simulink model "AIRCRAFT_ENGINE"  (Simulink 7.3)
settings: Solver=ode45  StartTime=0.0  StopTime=10.0  RelTol=1e-3
undefined symbols (not defined in the file): RootGround, RootPart
libraries: mblibv1 x68
settings Model: Creator=alvarez3  LastModifiedBy=congyue1
settings SimMechanicsCC: VisOnUpdateDiagram=on  VisDuringSimulation=on

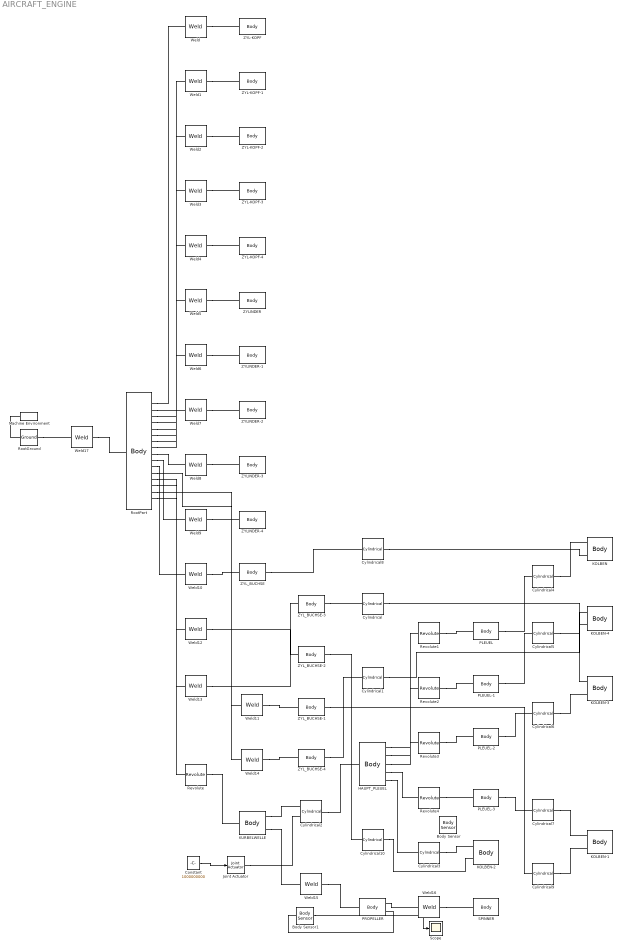
== system AIRCRAFT_ENGINE ==
  Body Sensor : mblibv1/Sensors &  Actuators/Body Sensor  DialogController=MECH.DynMechDlgSource  SystemSampleTime=-1  UpdateFromCAD=off  PhysicalDomain=Mechanical  PortType=blob  Muxed=on  Pose=off  Angle=on  AngleUnits=deg  ArcVelocity=off  ArcVelocityUnits=deg/s  ArcAcceleration=off  ArcAccelerationUnits=deg/s^2  CoordPosition=on  CoordPositionUnits=m  Velocity=off  VelocityUnits=m/s  Acceleration=off  AccelerationUnits=m/s^2  Quaternion=on  QuaternionDT=off  QuaternionDDT=off  QuaternionUnits=off  OutputVector=[1]  ActiveIO=off  Width=3  DialogClass=MechanicalSensorBlock  ReferenceFrame=Absolute (World)
  Body Sensor1 : mblibv1/Sensors &  Actuators/Body Sensor  DialogController=MECH.DynMechDlgSource  SystemSampleTime=-1  UpdateFromCAD=off  PhysicalDomain=Mechanical  PortType=blob  Muxed=on  Pose=on  Angle=on  AngleUnits=deg  ArcVelocity=off  ArcVelocityUnits=deg/s  ArcAcceleration=off  ArcAccelerationUnits=deg/s^2  CoordPosition=on  CoordPositionUnits=m  Velocity=off  VelocityUnits=m/s  Acceleration=off  AccelerationUnits=m/s^2  Quaternion=on  QuaternionDT=off  QuaternionDDT=off  QuaternionUnits=off  OutputVector=[1]  ActiveIO=on  Width=12  DialogClass=MechanicalSensorBlock  ReferenceFrame=Absolute (World)
  Constant : Constant  Value=1000000000  OutDataType=fixdt(1, 16)  OutScaling=2^0
  Cylindrical : mblibv1/Joints/Cylindrical  DialogController=MECH.DynMechDlgSource  PhysicalDomain=mechanical  SubClassName=Unknown  LeftPortType=blob  RightPortType=blob  LConnTagsString=__newl0  RConnTagsString=__newr0  PMImportedID=110:-:62  UpdateFromCAD=on  NumSAPorts=0  CutJoint=off  MarkAsCut=off  Primitives=prismatic  PrimitiveProps=P1$WORLD$[0,-0.309017,-0.951057]$prismatic#R1$WORLD$[0,0.309017,0.951057]$revolute  DialogClass=JointBlock  P1Axis=[0,-0.309017,-0.951057]  R1Axis=[0,0.309017,0.951057]
  Cylindrical1 : mblibv1/Joints/Cylindrical  DialogController=MECH.DynMechDlgSource  PhysicalDomain=mechanical  SubClassName=Unknown  LeftPortType=blob  RightPortType=blob  LConnTagsString=__newl0  RConnTagsString=__newr0  PMImportedID=81:-:89  UpdateFromCAD=on  NumSAPorts=0  CutJoint=off  MarkAsCut=off  Primitives=prismatic  PrimitiveProps=P1$WORLD$[0,0.809017,-0.587785]$prismatic#R1$WORLD$[0,-0.809017,0.587785]$revolute  DialogClass=JointBlock  P1Axis=[0,0.809017,-0.587785]  R1Axis=[0,-0.809017,0.587785]
  Cylindrical10 : mblibv1/Joints/Cylindrical  DialogController=MECH.DynMechDlgSource  PhysicalDomain=mechanical  SubClassName=Unknown  LeftPortType=blob  RightPortType=blob  LConnTagsString=__newl0  RConnTagsString=__newr0  PMImportedID=29:-:75  UpdateFromCAD=on  NumSAPorts=0  CutJoint=off  MarkAsCut=off  Primitives=prismatic  PrimitiveProps=P1$WORLD$[0,-0.309017,0.951057]$prismatic#R1$WORLD$[0,0.309017,-0.951057]$revolute  DialogClass=JointBlock  P1Axis=[0,-0.309017,0.951057]  R1Axis=[0,0.309017,-0.951057]
  Cylindrical2 : mblibv1/Joints/Cylindrical  DialogController=MECH.DynMechDlgSource  PhysicalDomain=mechanical  SubClassName=Unknown  LeftPortType=blob  RightPortType=blob  LConnTagsString=__newl0|SA1  RConnTagsString=__newr0  PMImportedID=74:-:76  UpdateFromCAD=on  NumSAPorts=1  CutJoint=off  MarkAsCut=off  Primitives=prismatic  PrimitiveProps=P1$World$[-1,0,0]$prismatic#R1$World$[1,0,0]$revolute  DialogClass=JointBlock  P1Axis=[-1,0,0]  R1Axis=[1,0,0]
  Cylindrical3 : mblibv1/Joints/Cylindrical  DialogController=MECH.DynMechDlgSource  PhysicalDomain=mechanical  SubClassName=Unknown  LeftPortType=blob  RightPortType=blob  LConnTagsString=__newl0  RConnTagsString=__newr0  PMImportedID=74:-:75  UpdateFromCAD=on  NumSAPorts=0  CutJoint=off  MarkAsCut=off  Primitives=prismatic  PrimitiveProps=P1$WORLD$[1,0,0]$prismatic#R1$WORLD$[-1,0,0]$revolute  DialogClass=JointBlock  P1Axis=[1,0,0]  R1Axis=[-1,0,0]
  Cylindrical4 : mblibv1/Joints/Cylindrical  DialogController=MECH.DynMechDlgSource  PhysicalDomain=mechanical  SubClassName=Unknown  LeftPortType=blob  RightPortType=blob  LConnTagsString=__newl0  RConnTagsString=__newr0  PMImportedID=106:-:79  UpdateFromCAD=on  NumSAPorts=0  CutJoint=off  MarkAsCut=off  Primitives=prismatic  PrimitiveProps=P1$WORLD$[1,0,0]$prismatic#R1$WORLD$[1,0,0]$revolute  DialogClass=JointBlock  P1Axis=[1,0,0]  R1Axis=[1,0,0]
  Cylindrical5 : mblibv1/Joints/Cylindrical  DialogController=MECH.DynMechDlgSource  PhysicalDomain=mechanical  SubClassName=Unknown  LeftPortType=blob  RightPortType=blob  LConnTagsString=__newl0  RConnTagsString=__newr0  PMImportedID=108:-:81  UpdateFromCAD=on  NumSAPorts=0  CutJoint=off  MarkAsCut=off  Primitives=prismatic  PrimitiveProps=P1$WORLD$[1,0,0]$prismatic#R1$WORLD$[-1,0,0]$revolute  DialogClass=JointBlock  P1Axis=[1,0,0]  R1Axis=[-1,0,0]
  Cylindrical6 : mblibv1/Joints/Cylindrical  DialogController=MECH.DynMechDlgSource  PhysicalDomain=mechanical  SubClassName=Unknown  LeftPortType=blob  RightPortType=blob  LConnTagsString=__newl0  RConnTagsString=__newr0  PMImportedID=110:-:113  UpdateFromCAD=on  NumSAPorts=0  CutJoint=off  MarkAsCut=off  Primitives=prismatic  PrimitiveProps=P1$WORLD$[1,0,0]$prismatic#R1$WORLD$[1,0,0]$revolute  DialogClass=JointBlock  P1Axis=[1,0,0]  R1Axis=[1,0,0]
  Cylindrical7 : mblibv1/Joints/Cylindrical  DialogController=MECH.DynMechDlgSource  PhysicalDomain=mechanical  SubClassName=Unknown  LeftPortType=blob  RightPortType=blob  LConnTagsString=__newl0  RConnTagsString=__newr0  PMImportedID=104:-:73  UpdateFromCAD=on  NumSAPorts=0  CutJoint=off  MarkAsCut=off  Primitives=prismatic  PrimitiveProps=P1$WORLD$[1,0,0]$prismatic#R1$WORLD$[1,0,0]$revolute  DialogClass=JointBlock  P1Axis=[1,0,0]  R1Axis=[1,0,0]
  Cylindrical8 : mblibv1/Joints/Cylindrical  DialogController=MECH.DynMechDlgSource  PhysicalDomain=mechanical  SubClassName=Unknown  LeftPortType=blob  RightPortType=blob  LConnTagsString=__newl0  RConnTagsString=__newr0  PMImportedID=106:-:42  UpdateFromCAD=on  NumSAPorts=0  CutJoint=off  MarkAsCut=off  Primitives=prismatic  PrimitiveProps=P1$WORLD$[0,0.809017,0.587785]$prismatic#R1$WORLD$[0,-0.809017,-0.587785]$revolute  DialogClass=JointBlock  P1Axis=[0,0.809017,0.587785]  R1Axis=[0,-0.809017,-0.587785]
  Cylindrical9 : mblibv1/Joints/Cylindrical  DialogController=MECH.DynMechDlgSource  PhysicalDomain=mechanical  SubClassName=Unknown  LeftPortType=blob  RightPortType=blob  LConnTagsString=__newl0  RConnTagsString=__newr0  PMImportedID=18:-:73  UpdateFromCAD=on  NumSAPorts=0  CutJoint=off  MarkAsCut=off  Primitives=prismatic  PrimitiveProps=P1$WORLD$[0,-1,0]$prismatic#R1$WORLD$[0,1,0]$revolute  DialogClass=JointBlock  P1Axis=[0,-1,0]  R1Axis=[0,1,0]
  HAUPT_PLEUEL : mblibv1/Bodies/Body  DialogController=MECH.DynMechDlgSource  PhysicalDomain=mechanical  SubClassName=Unknown  LeftPortType=workingframe  RightPortType=workingframe  LConnTagsString=CS2  RConnTagsString=CS3|CS4|CS5|CS6|CS7  PMImportedID=74  UpdateFromCAD=on  DialogClass=MechanicalBodyBlock  Mass=1.80809e+007  MassUnits=kg  InertiaUnits=kg*m^2  Inertia=[2281.27,0,0;0,8743.05,0;0,0,10016.5]  Shape=Cylinder  ShapeDims=[1 1]  ShapeUnits=m  ShapeUse=false  Density=1  DensityUnits=kg/m^3  DensityUse=false  GraphicsMode=GFXFILE  GraphicsFileName=HAUPT_PLEUEL_prt.stl  BodyColorSelMode=MACHINE_DEFAULT  BodyColor=[1 0 0]  AttachedToCS=CS1  CG=Right$CG$[-20.2 0.0648404 0.83431]$WORLD$WORLD$mm$[0 0 -1;-0.303086 0.952963 0;0.952963 0.303086 0]$3x3 Transform$rad$WORLD$false$74::CG(AUTOGEN)  WorkingFrames=Right$CS1$[-20.2 9.54534 -28.9743]$WORLD$WORLD$mm$[0 0 -1;-0.303086 0.952963 0;0.952963 0.303086 0]$3x3 Transform$rad$WORLD$false$74::CS1(AUTOGEN)#Left$CS2$[-33.05 -3.03256 10.5737]$WORLD$WORLD$mm$[1 0 0;0 1 0;0 0 1]$3x3 Transform$rad$WORLD$true$74:-:76::74(AUTOGEN)#Right$CS3$[-15.2998 -19.2856 -1.08076]$WORLD$WORLD$mm$[1 0 0;0 1 0;0 0 1]$3x3 Transform$rad$WORLD$true$74:-:79::74(AUTOGEN)#Right$CS4$[-29 -19.1395 22.43]$WORLD$WORLD$mm$[1 0 0;0 1 0;0 0 1]$3x3 Transform$rad$WORLD$true$108:-:74::74(AUTOGEN)#Right$CS5$[-25.1002 3.26616 29.556]$WORLD$WORLD$mm$[1 0 0;0 1 0;0 0 1]$3x3 Transform$rad$WORLD$true$113:-:74::74(AUTOGEN)#Right$CS6$[-29 16.9669 10.4491]$WORLD$WORLD$mm$[1 0 0;0 1 0;0 0 1]$3x3 Transform$rad$WORLD$true$104:-:74::74(AUTOGEN)#Right$CS7$[-15.3 15.6071 -48.0336]$WORLD$WORLD$mm$[1 0 0;0 1 0;0 0 1]$3x3 Transform$rad$WORLD$true$74:-:75::74(AUTOGEN)  CGPos=[-20.2 0.0648404 0.83431]  CGRot=[0 0 -1;-0.303086 0.952963 0;0.952963 0.303086 0]  CS0Pos=[]  CS0Rot=[]  CS1Pos=[-20.2 9.54534 -28.9743]  CS1Rot=[0 0 -1;-0.303086 0.952963 0;0.952963 0.303086 0]  CS2Pos=[-33.05 -3.03256 10.5737]  CS2Rot=[1 0 0;0 1 0;0 0 1]  CS3Pos=[-15.2998 -19.2856 -1.08076]  CS3Rot=[1 0 0;0 1 0;0 0 1]  CS4Pos=[-29 -19.1395 22.43]  CS4Rot=[1 0 0;0 1 0;0 0 1]  CS5Pos=[-25.1002 3.26616 29.556]  CS5Rot=[1 0 0;0 1 0;0 0 1]  CS6Pos=[-29 16.9669 10.4491]  CS6Rot=[1 0 0;0 1 0;0 0 1]  CS7Pos=[-15.3 15.6071 -48.0336]  CS7Rot=[1 0 0;0 1 0;0 0 1]  CS8Pos=[]  CS8Rot=[]  CS9Pos=[]  CS9Rot=[]  CS10Pos=[]  CS10Rot=[]  CS11Pos=[]  CS11Rot=[]  CS12Pos=[]  CS12Rot=[]  CS13Pos=[]  CS13Rot=[]  CS14Pos=[]  CS14Rot=[]  CS15Pos=[]  CS15Rot=[]  CS16Pos=[]  CS16Rot=[]  CS17Pos=[]  CS17Rot=[]  CS18Pos=[]  CS18Rot=[]  CS19Pos=[]  CS19Rot=[]  CS20Pos=[]  CS20Rot=[]
  Joint Actuator : mblibv1/Sensors &  Actuators/Joint Actuator  DialogController=MECH.DynMechDlgSource  SystemSampleTime=-1  UpdateFromCAD=off  PhysicalDomain=Mechanical  PortType=blob  ActuationStyle=Force  AngleUnits=deg  ArcVelocityUnits=deg/s  ArcAccelerationUnits=deg/s^2  CoordPositionUnits=m  VelocityUnits=m/s  AccelerationUnits=m/s^2  ForceUnits=N  TorqueUnits=N*m  ActiveIO=on  Width=1  DialogClass=MechanicalActuatorBlock  Primitive=R1  ReferenceFrame=Absolute (World)
  KOLBEN : mblibv1/Bodies/Body  DialogController=MECH.DynMechDlgSource  PhysicalDomain=mechanical  SubClassName=Unknown  LeftPortType=workingframe  RightPortType=workingframe  LConnTagsString=CS2|CS3  PMImportedID=106  UpdateFromCAD=on  DialogClass=MechanicalBodyBlock  Mass=4.9128e+006  MassUnits=kg  InertiaUnits=kg*m^2  Inertia=[374.226,0,0;0,458.442,0;0,0,380.048]  Shape=Cylinder  ShapeDims=[1 1]  ShapeUnits=m  ShapeUse=false  Density=1  DensityUnits=kg/m^3  DensityUse=false  GraphicsMode=GFXFILE  GraphicsFileName=KOLBEN_prt.stl  BodyColorSelMode=MACHINE_DEFAULT  BodyColor=[1 0 0]  AttachedToCS=CS1  CG=Right$CG$[-25 -48.5239 -35.2546]$WORLD$WORLD$mm$[1 0 0;0 0.809017 -0.587785;0 0.587785 0.809017]$3x3 Transform$rad$WORLD$false$106::CG(AUTOGEN)  WorkingFrames=Right$CS1$[-25 -55.3483 -40.2129]$WORLD$WORLD$mm$[1 0 0;0 0.809017 -0.587785;0 0.587785 0.809017]$3x3 Transform$rad$WORLD$false$106::CS1(AUTOGEN)#Left$CS2$[-25.1 -46.0446 -33.4533]$WORLD$WORLD$mm$[1 0 0;0 1 0;0 0 1]$3x3 Transform$rad$WORLD$true$106:-:79::106(AUTOGEN)#Left$CS3$[-25 -33.5491 -24.3749]$WORLD$WORLD$mm$[1 0 0;0 1 0;0 0 1]$3x3 Transform$rad$WORLD$true$106:-:42::106(AUTOGEN)  CGPos=[-25 -48.5239 -35.2546]  CGRot=[1 0 0;0 0.809017 -0.587785;0 0.587785 0.809017]  CS0Pos=[]  CS0Rot=[]  CS1Pos=[-25 -55.3483 -40.2129]  CS1Rot=[1 0 0;0 0.809017 -0.587785;0 0.587785 0.809017]  CS2Pos=[-25.1 -46.0446 -33.4533]  CS2Rot=[1 0 0;0 1 0;0 0 1]  CS3Pos=[-25 -33.5491 -24.3749]  CS3Rot=[1 0 0;0 1 0;0 0 1]  CS4Pos=[]  CS4Rot=[]  CS5Pos=[]  CS5Rot=[]  CS6Pos=[]  CS6Rot=[]  CS7Pos=[]  CS7Rot=[]  CS8Pos=[]  CS8Rot=[]  CS9Pos=[]  CS9Rot=[]  CS10Pos=[]  CS10Rot=[]  CS11Pos=[]  CS11Rot=[]  CS12Pos=[]  CS12Rot=[]  CS13Pos=[]  CS13Rot=[]  CS14Pos=[]  CS14Rot=[]  CS15Pos=[]  CS15Rot=[]  CS16Pos=[]  CS16Rot=[]  CS17Pos=[]  CS17Rot=[]  CS18Pos=[]  CS18Rot=[]  CS19Pos=[]  CS19Rot=[]  CS20Pos=[]  CS20Rot=[]
  KOLBEN-1 : mblibv1/Bodies/Body  DialogController=MECH.DynMechDlgSource  PhysicalDomain=mechanical  SubClassName=Unknown  LeftPortType=workingframe  RightPortType=workingframe  LConnTagsString=CS2|CS3  PMImportedID=73  UpdateFromCAD=on  DialogClass=MechanicalBodyBlock  Mass=4.9128e+006  MassUnits=kg  InertiaUnits=kg*m^2  Inertia=[374.226,0,0;0,458.442,0;0,0,380.048]  Shape=Cylinder  ShapeDims=[1 1]  ShapeUnits=m  ShapeUse=false  Density=1  DensityUnits=kg/m^3  DensityUse=false  GraphicsMode=GFXFILE  GraphicsFileName=KOLBEN_prt.stl  BodyColorSelMode=MACHINE_DEFAULT  BodyColor=[1 0 0]  AttachedToCS=CS1  CG=Right$CG$[-25 60.711 0]$WORLD$WORLD$mm$[1 0 0;0 -1 0;0 0 -1]$3x3 Transform$rad$WORLD$false$73::CG(AUTOGEN)  WorkingFrames=Right$CS1$[-25 69.1465 0]$WORLD$WORLD$mm$[1 0 0;0 -1 0;0 0 -1]$3x3 Transform$rad$WORLD$false$73::CS1(AUTOGEN)#Left$CS2$[-25.1 57.6465 0]$WORLD$WORLD$mm$[1 0 0;0 1 0;0 0 1]$3x3 Transform$rad$WORLD$true$104:-:73::73(AUTOGEN)#Left$CS3$[-25 41.469 0]$WORLD$WORLD$mm$[1 0 0;0 1 0;0 0 1]$3x3 Transform$rad$WORLD$true$18:-:73::73(AUTOGEN)  CGPos=[-25 60.711 0]  CGRot=[1 0 0;0 -1 0;0 0 -1]  CS0Pos=[]  CS0Rot=[]  CS1Pos=[-25 69.1465 0]  CS1Rot=[1 0 0;0 -1 0;0 0 -1]  CS2Pos=[-25.1 57.6465 0]  CS2Rot=[1 0 0;0 1 0;0 0 1]  CS3Pos=[-25 41.469 0]  CS3Rot=[1 0 0;0 1 0;0 0 1]  CS4Pos=[]  CS4Rot=[]  CS5Pos=[]  CS5Rot=[]  CS6Pos=[]  CS6Rot=[]  CS7Pos=[]  CS7Rot=[]  CS8Pos=[]  CS8Rot=[]  CS9Pos=[]  CS9Rot=[]  CS10Pos=[]  CS10Rot=[]  CS11Pos=[]  CS11Rot=[]  CS12Pos=[]  CS12Rot=[]  CS13Pos=[]  CS13Rot=[]  CS14Pos=[]  CS14Rot=[]  CS15Pos=[]  CS15Rot=[]  CS16Pos=[]  CS16Rot=[]  CS17Pos=[]  CS17Rot=[]  CS18Pos=[]  CS18Rot=[]  CS19Pos=[]  CS19Rot=[]  CS20Pos=[]  CS20Rot=[]
  KOLBEN-2 : mblibv1/Bodies/Body  DialogController=MECH.DynMechDlgSource  PhysicalDomain=mechanical  SubClassName=Unknown  LeftPortType=workingframe  RightPortType=workingframe  LConnTagsString=CS2|CS3  PMImportedID=75  UpdateFromCAD=on  DialogClass=MechanicalBodyBlock  Mass=4.9128e+006  MassUnits=kg  InertiaUnits=kg*m^2  Inertia=[374.226,0,0;0,458.442,0;0,0,380.048]  Shape=Cylinder  ShapeDims=[1 1]  ShapeUnits=m  ShapeUse=false  Density=1  DensityUnits=kg/m^3  DensityUse=false  GraphicsMode=GFXFILE  GraphicsFileName=KOLBEN_prt.stl  BodyColorSelMode=MACHINE_DEFAULT  BodyColor=[1 0 0]  AttachedToCS=CS1  CG=Right$CG$[-25 16.5541 -50.9481]$WORLD$WORLD$mm$[1 0 0;0 -0.309017 -0.951057;0 0.951057 -0.309017]$3x3 Transform$rad$WORLD$false$75::CG(AUTOGEN)  WorkingFrames=Right$CS1$[-25 19.1607 -58.9707]$WORLD$WORLD$mm$[1 0 0;0 -0.309017 -0.951057;0 0.951057 -0.309017]$3x3 Transform$rad$WORLD$false$75::CS1(AUTOGEN)#Left$CS2$[-15.3 15.6071 -48.0336]$WORLD$WORLD$mm$[1 0 0;0 1 0;0 0 1]$3x3 Transform$rad$WORLD$true$74:-:75::75(AUTOGEN)#Left$CS3$[-25 12.8146 -39.4393]$WORLD$WORLD$mm$[1 0 0;0 1 0;0 0 1]$3x3 Transform$rad$WORLD$true$29:-:75::75(AUTOGEN)  CGPos=[-25 16.5541 -50.9481]  CGRot=[1 0 0;0 -0.309017 -0.951057;0 0.951057 -0.309017]  CS0Pos=[]  CS0Rot=[]  CS1Pos=[-25 19.1607 -58.9707]  CS1Rot=[1 0 0;0 -0.309017 -0.951057;0 0.951057 -0.309017]  CS2Pos=[-15.3 15.6071 -48.0336]  CS2Rot=[1 0 0;0 1 0;0 0 1]  CS3Pos=[-25 12.8146 -39.4393]  CS3Rot=[1 0 0;0 1 0;0 0 1]  CS4Pos=[]  CS4Rot=[]  CS5Pos=[]  CS5Rot=[]  CS6Pos=[]  CS6Rot=[]  CS7Pos=[]  CS7Rot=[]  CS8Pos=[]  CS8Rot=[]  CS9Pos=[]  CS9Rot=[]  CS10Pos=[]  CS10Rot=[]  CS11Pos=[]  CS11Rot=[]  CS12Pos=[]  CS12Rot=[]  CS13Pos=[]  CS13Rot=[]  CS14Pos=[]  CS14Rot=[]  CS15Pos=[]  CS15Rot=[]  CS16Pos=[]  CS16Rot=[]  CS17Pos=[]  CS17Rot=[]  CS18Pos=[]  CS18Rot=[]  CS19Pos=[]  CS19Rot=[]  CS20Pos=[]  CS20Rot=[]
  KOLBEN-3 : mblibv1/Bodies/Body  DialogController=MECH.DynMechDlgSource  PhysicalDomain=mechanical  SubClassName=Unknown  LeftPortType=workingframe  RightPortType=workingframe  LConnTagsString=CS2|CS3  PMImportedID=110  UpdateFromCAD=on  DialogClass=MechanicalBodyBlock  Mass=4.9128e+006  MassUnits=kg  InertiaUnits=kg*m^2  Inertia=[374.226,0,0;0,458.442,0;0,0,380.048]  Shape=Cylinder  ShapeDims=[1 1]  ShapeUnits=m  ShapeUse=false  Density=1  DensityUnits=kg/m^3  DensityUse=false  GraphicsMode=GFXFILE  GraphicsFileName=KOLBEN_prt.stl  BodyColorSelMode=MACHINE_DEFAULT  BodyColor=[1 0 0]  AttachedToCS=CS1  CG=Right$CG$[-25 22.7896 70.1391]$WORLD$WORLD$mm$[1 0 0;0 -0.309017 0.951057;0 -0.951057 -0.309017]$3x3 Transform$rad$WORLD$false$110::CG(AUTOGEN)  WorkingFrames=Right$CS1$[-25 25.3963 78.1616]$WORLD$WORLD$mm$[1 0 0;0 -0.309017 0.951057;0 -0.951057 -0.309017]$3x3 Transform$rad$WORLD$false$110::CS1(AUTOGEN)#Left$CS2$[-25 12.8146 39.4393]$WORLD$WORLD$mm$[1 0 0;0 1 0;0 0 1]$3x3 Transform$rad$WORLD$true$110:-:62::110(AUTOGEN)#Left$CS3$[-25.1 21.8426 67.2245]$WORLD$WORLD$mm$[1 0 0;0 1 0;0 0 1]$3x3 Transform$rad$WORLD$true$110:-:113::110(AUTOGEN)  CGPos=[-25 22.7896 70.1391]  CGRot=[1 0 0;0 -0.309017 0.951057;0 -0.951057 -0.309017]  CS0Pos=[]  CS0Rot=[]  CS1Pos=[-25 25.3963 78.1616]  CS1Rot=[1 0 0;0 -0.309017 0.951057;0 -0.951057 -0.309017]  CS2Pos=[-25 12.8146 39.4393]  CS2Rot=[1 0 0;0 1 0;0 0 1]  CS3Pos=[-25.1 21.8426 67.2245]  CS3Rot=[1 0 0;0 1 0;0 0 1]  CS4Pos=[]  CS4Rot=[]  CS5Pos=[]  CS5Rot=[]  CS6Pos=[]  CS6Rot=[]  CS7Pos=[]  CS7Rot=[]  CS8Pos=[]  CS8Rot=[]  CS9Pos=[]  CS9Rot=[]  CS10Pos=[]  CS10Rot=[]  CS11Pos=[]  CS11Rot=[]  CS12Pos=[]  CS12Rot=[]  CS13Pos=[]  CS13Rot=[]  CS14Pos=[]  CS14Rot=[]  CS15Pos=[]  CS15Rot=[]  CS16Pos=[]  CS16Rot=[]  CS17Pos=[]  CS17Rot=[]  CS18Pos=[]  CS18Rot=[]  CS19Pos=[]  CS19Rot=[]  CS20Pos=[]  CS20Rot=[]
  KOLBEN-4 : mblibv1/Bodies/Body  DialogController=MECH.DynMechDlgSource  PhysicalDomain=mechanical  SubClassName=Unknown  LeftPortType=workingframe  RightPortType=workingframe  LConnTagsString=CS2|CS3  PMImportedID=81  UpdateFromCAD=on  DialogClass=MechanicalBodyBlock  Mass=4.9128e+006  MassUnits=kg  InertiaUnits=kg*m^2  Inertia=[374.226,0,0;0,458.442,0;0,0,380.048]  Shape=Cylinder  ShapeDims=[1 1]  ShapeUnits=m  ShapeUse=false  Density=1  DensityUnits=kg/m^3  DensityUse=false  GraphicsMode=GFXFILE  GraphicsFileName=KOLBEN_prt.stl  BodyColorSelMode=MACHINE_DEFAULT  BodyColor=[1 0 0]  AttachedToCS=CS1  CG=Right$CG$[-25 -59.1898 43.0039]$WORLD$WORLD$mm$[1 0 0;0 0.809017 0.587785;0 -0.587785 0.809017]$3x3 Transform$rad$WORLD$false$81::CG(AUTOGEN)  WorkingFrames=Right$CS1$[-25 -66.0142 47.9621]$WORLD$WORLD$mm$[1 0 0;0 0.809017 0.587785;0 -0.587785 0.809017]$3x3 Transform$rad$WORLD$false$81::CS1(AUTOGEN)#Left$CS2$[-25 -33.5491 24.3749]$WORLD$WORLD$mm$[1 0 0;0 1 0;0 0 1]$3x3 Transform$rad$WORLD$true$81:-:89::81(AUTOGEN)#Left$CS3$[-15.3 -56.7105 41.2026]$WORLD$WORLD$mm$[1 0 0;0 1 0;0 0 1]$3x3 Transform$rad$WORLD$true$108:-:81::81(AUTOGEN)  CGPos=[-25 -59.1898 43.0039]  CGRot=[1 0 0;0 0.809017 0.587785;0 -0.587785 0.809017]  CS0Pos=[]  CS0Rot=[]  CS1Pos=[-25 -66.0142 47.9621]  CS1Rot=[1 0 0;0 0.809017 0.587785;0 -0.587785 0.809017]  CS2Pos=[-25 -33.5491 24.3749]  CS2Rot=[1 0 0;0 1 0;0 0 1]  CS3Pos=[-15.3 -56.7105 41.2026]  CS3Rot=[1 0 0;0 1 0;0 0 1]  CS4Pos=[]  CS4Rot=[]  CS5Pos=[]  CS5Rot=[]  CS6Pos=[]  CS6Rot=[]  CS7Pos=[]  CS7Rot=[]  CS8Pos=[]  CS8Rot=[]  CS9Pos=[]  CS9Rot=[]  CS10Pos=[]  CS10Rot=[]  CS11Pos=[]  CS11Rot=[]  CS12Pos=[]  CS12Rot=[]  CS13Pos=[]  CS13Rot=[]  CS14Pos=[]  CS14Rot=[]  CS15Pos=[]  CS15Rot=[]  CS16Pos=[]  CS16Rot=[]  CS17Pos=[]  CS17Rot=[]  CS18Pos=[]  CS18Rot=[]  CS19Pos=[]  CS19Rot=[]  CS20Pos=[]  CS20Rot=[]
  KURBELWELLE : mblibv1/Bodies/Body  DialogController=MECH.DynMechDlgSource  PhysicalDomain=mechanical  SubClassName=Unknown  LeftPortType=workingframe  RightPortType=workingframe  LConnTagsString=CS4  RConnTagsString=CS2|CS3  PMImportedID=76  UpdateFromCAD=on  DialogClass=MechanicalBodyBlock  Mass=3.09e+007  MassUnits=kg  InertiaUnits=kg*m^2  Inertia=[5969.93,-2644.36,0;-2644.36,31773.2,0;0,0,31794]  Shape=Cylinder  ShapeDims=[1 1]  ShapeUnits=m  ShapeUse=false  Density=1  DensityUnits=kg/m^3  DensityUse=false  GraphicsMode=GFXFILE  GraphicsFileName=KURBELWELLE_prt.stl  BodyColorSelMode=MACHINE_DEFAULT  BodyColor=[1 0 0]  AttachedToCS=CS1  CG=Right$CG$[12.4062 1.16057 -4.0466]$WORLD$WORLD$mm$[1 0 0;0 -0.275687 -0.961247;0 0.961247 -0.275687]$3x3 Transform$rad$WORLD$false$76::CG(AUTOGEN)  WorkingFrames=Right$CS1$[17.45 0 0]$WORLD$WORLD$mm$[1 0 0;0 -0.275687 -0.961247;0 0.961247 -0.275687]$3x3 Transform$rad$WORLD$false$76::CS1(AUTOGEN)#Right$CS2$[-33.05 -3.03256 10.5737]$WORLD$WORLD$mm$[1 0 0;0 1 0;0 0 1]$3x3 Transform$rad$WORLD$true$74:-:76::76(AUTOGEN)#Right$CS3$[90.95 0 0]$WORLD$WORLD$mm$[1 0 0;0 1 0;0 0 1]$3x3 Transform$rad$WORLD$true$111:-:76::76(AUTOGEN)#Left$CS4$[-5.05 0 0]$WORLD$WORLD$mm$[1 0 0;0 1 0;0 0 1]$3x3 Transform$rad$WORLD$true$:-:RootPart::76(AUTOGEN)  CGPos=[12.4062 1.16057 -4.0466]  CGRot=[1 0 0;0 -0.275687 -0.961247;0 0.961247 -0.275687]  CS0Pos=[]  CS0Rot=[]  CS1Pos=[17.45 0 0]  CS1Rot=[1 0 0;0 -0.275687 -0.961247;0 0.961247 -0.275687]  CS2Pos=[-33.05 -3.03256 10.5737]  CS2Rot=[1 0 0;0 1 0;0 0 1]  CS3Pos=[90.95 0 0]  CS3Rot=[1 0 0;0 1 0;0 0 1]  CS4Pos=[-5.05 0 0]  CS4Rot=[1 0 0;0 1 0;0 0 1]  CS5Pos=[]  CS5Rot=[]  CS6Pos=[]  CS6Rot=[]  CS7Pos=[]  CS7Rot=[]  CS8Pos=[]  CS8Rot=[]  CS9Pos=[]  CS9Rot=[]  CS10Pos=[]  CS10Rot=[]  CS11Pos=[]  CS11Rot=[]  CS12Pos=[]  CS12Rot=[]  CS13Pos=[]  CS13Rot=[]  CS14Pos=[]  CS14Rot=[]  CS15Pos=[]  CS15Rot=[]  CS16Pos=[]  CS16Rot=[]  CS17Pos=[]  CS17Rot=[]  CS18Pos=[]  CS18Rot=[]  CS19Pos=[]  CS19Rot=[]  CS20Pos=[]  CS20Rot=[]
  Machine Environment : mblibv1/Bodies/Machine Environment  DialogController=MECH.DialogSource  SystemSampleTime=-1  PortType=env  PhysicalDomain=Mechanical  DialogTemplateClass=MECH.MachineEnvironment  SyncWhenCopied=off  Gravity=[0 -9.81 0]  GravityUnits=m/s^2  GravityAsSignal=off  Dimensionality=Auto-detect  AnalysisType=Forward dynamics  LinearAssemblyTolerance=1e-3  LinearAssemblyToleranceUnits=m  AngularAssemblyTolerance=1e-3  AngularAssemblyToleranceUnits=rad  ConstraintSolverType=Stabilizing  ConstraintRelTolerance=1e-4  ConstraintAbsTolerance=1e-4  UseRobustSingularityHandling=off  RedundancyAnalysisToleranceType=Automatically select tolerance  RedundancyAnalysisTolerance=1e-14  StatePerturbationType=Fixed  PerturbationSize=1e-5  VisualizeMachine=on  BodyVisualizationType=Use model default body geometries  BodyColorSelMode=Use model default  DefaultBodyColor=[1 0 0]
  PLEUEL : mblibv1/Bodies/Body  DialogController=MECH.DynMechDlgSource  PhysicalDomain=mechanical  SubClassName=Unknown  LeftPortType=workingframe  RightPortType=workingframe  LConnTagsString=CS2  RConnTagsString=CS3  PMImportedID=79  UpdateFromCAD=on  DialogClass=MechanicalBodyBlock  Mass=4.9128e+006  MassUnits=kg  InertiaUnits=kg*m^2  Inertia=[14.226,0,0;0,458.442,0;0,0,380.048]  Shape=Cylinder  ShapeDims=[1 1]  ShapeUnits=m  ShapeUse=false  Density=1  DensityUnits=kg/m^3  DensityUse=false  GraphicsMode=GFXFILE  GraphicsFileName=C:\Documents and Settings\alvarez3\Desktop\test\pleuel_prt.stl  BodyColorSelMode=MACHINE_DEFAULT  BodyColor=[1 0 0]  AttachedToCS=CS1  CG=Right$CG$[-20.2 -32.6652 -17.2671]$WORLD$WORLD$mm$[0 0 1;-0.637111 0.770772 0;-0.770772 -0.637111 0]$3x3 Transform$rad$WORLD$false$79::CG(AUTOGEN)  WorkingFrames=Right$CS1$[-20.2 -32.6652 -17.2671]$WORLD$WORLD$mm$[0 0 1;-0.637111 0.770772 0;-0.770772 -0.637111 0]$3x3 Transform$rad$WORLD$false$79::CS1(AUTOGEN)#Left$CS2$[-15.2998 -19.2856 -1.08076]$WORLD$WORLD$mm$[1 0 0;0 1 0;0 0 1]$3x3 Transform$rad$WORLD$true$74:-:79::79(AUTOGEN)#Right$CS3$[-25.1 -46.0446 -33.4533]$WORLD$WORLD$mm$[1 0 0;0 1 0;0 0 1]$3x3 Transform$rad$WORLD$true$106:-:79::79(AUTOGEN)  CGPos=[-20.2 -32.6652 -17.2671]  CGRot=[0 0 1;-0.637111 0.770772 0;-0.770772 -0.637111 0]  CS0Pos=[]  CS0Rot=[]  CS1Pos=[-20.2 -32.6652 -17.2671]  CS1Rot=[0 0 1;-0.637111 0.770772 0;-0.770772 -0.637111 0]  CS2Pos=[-15.2998 -19.2856 -1.08076]  CS2Rot=[1 0 0;0 1 0;0 0 1]  CS3Pos=[-25.1 -46.0446 -33.4533]  CS3Rot=[1 0 0;0 1 0;0 0 1]  CS4Pos=[]  CS4Rot=[]  CS5Pos=[]  CS5Rot=[]  CS6Pos=[]  CS6Rot=[]  CS7Pos=[]  CS7Rot=[]  CS8Pos=[]  CS8Rot=[]  CS9Pos=[]  CS9Rot=[]  CS10Pos=[]  CS10Rot=[]  CS11Pos=[]  CS11Rot=[]  CS12Pos=[]  CS12Rot=[]  CS13Pos=[]  CS13Rot=[]  CS14Pos=[]  CS14Rot=[]  CS15Pos=[]  CS15Rot=[]  CS16Pos=[]  CS16Rot=[]  CS17Pos=[]  CS17Rot=[]  CS18Pos=[]  CS18Rot=[]  CS19Pos=[]  CS19Rot=[]  CS20Pos=[]  CS20Rot=[]
  PLEUEL-1 : mblibv1/Bodies/Body  DialogController=MECH.DynMechDlgSource  PhysicalDomain=mechanical  SubClassName=Unknown  LeftPortType=workingframe  RightPortType=workingframe  LConnTagsString=CS2  RConnTagsString=CS3  PMImportedID=108  UpdateFromCAD=on  DialogClass=MechanicalBodyBlock  Mass=4.9128e+006  MassUnits=kg  InertiaUnits=kg*m^2  Inertia=[14.226,0,0;0,458.442,0;0,0,380.048]  Shape=Cylinder  ShapeDims=[1 1]  ShapeUnits=m  ShapeUse=false  Density=1  DensityUnits=kg/m^3  DensityUse=false  GraphicsMode=GFXFILE  GraphicsFileName=PLEUEL_prt.stl  BodyColorSelMode=MACHINE_DEFAULT  BodyColor=[1 0 0]  AttachedToCS=CS1  CG=Right$CG$[-20.2 -37.9249 31.8163]$WORLD$WORLD$mm$[0 0 -1;0.894551 -0.446966 0;-0.446966 -0.894551 0]$3x3 Transform$rad$WORLD$false$108::CG(AUTOGEN)  WorkingFrames=Right$CS1$[-20.2 -37.9249 31.8163]$WORLD$WORLD$mm$[0 0 -1;0.894551 -0.446966 0;-0.446966 -0.894551 0]$3x3 Transform$rad$WORLD$false$108::CS1(AUTOGEN)#Left$CS2$[-29 -19.1395 22.43]$WORLD$WORLD$mm$[1 0 0;0 1 0;0 0 1]$3x3 Transform$rad$WORLD$true$108:-:74::108(AUTOGEN)#Right$CS3$[-15.3 -56.7105 41.2026]$WORLD$WORLD$mm$[1 0 0;0 1 0;0 0 1]$3x3 Transform$rad$WORLD$true$108:-:81::108(AUTOGEN)  CGPos=[-20.2 -37.9249 31.8163]  CGRot=[0 0 -1;0.894551 -0.446966 0;-0.446966 -0.894551 0]  CS0Pos=[]  CS0Rot=[]  CS1Pos=[-20.2 -37.9249 31.8163]  CS1Rot=[0 0 -1;0.894551 -0.446966 0;-0.446966 -0.894551 0]  CS2Pos=[-29 -19.1395 22.43]  CS2Rot=[1 0 0;0 1 0;0 0 1]  CS3Pos=[-15.3 -56.7105 41.2026]  CS3Rot=[1 0 0;0 1 0;0 0 1]  CS4Pos=[]  CS4Rot=[]  CS5Pos=[]  CS5Rot=[]  CS6Pos=[]  CS6Rot=[]  CS7Pos=[]  CS7Rot=[]  CS8Pos=[]  CS8Rot=[]  CS9Pos=[]  CS9Rot=[]  CS10Pos=[]  CS10Rot=[]  CS11Pos=[]  CS11Rot=[]  CS12Pos=[]  CS12Rot=[]  CS13Pos=[]  CS13Rot=[]  CS14Pos=[]  CS14Rot=[]  CS15Pos=[]  CS15Rot=[]  CS16Pos=[]  CS16Rot=[]  CS17Pos=[]  CS17Rot=[]  CS18Pos=[]  CS18Rot=[]  CS19Pos=[]  CS19Rot=[]  CS20Pos=[]  CS20Rot=[]
  PLEUEL-2 : mblibv1/Bodies/Body  DialogController=MECH.DynMechDlgSource  PhysicalDomain=mechanical  SubClassName=Unknown  LeftPortType=workingframe  RightPortType=workingframe  LConnTagsString=CS2  RConnTagsString=CS3  PMImportedID=113  UpdateFromCAD=on  DialogClass=MechanicalBodyBlock  Mass=4.9128e+006  MassUnits=kg  InertiaUnits=kg*m^2  Inertia=[14.226,0,0;0,458.442,0;0,0,380.048]  Shape=Cylinder  ShapeDims=[1 1]  ShapeUnits=m  ShapeUse=false  Density=1  DensityUnits=kg/m^3  DensityUse=false  GraphicsMode=GFXFILE  GraphicsFileName=PLEUEL_prt.stl  BodyColorSelMode=MACHINE_DEFAULT  BodyColor=[1 0 0]  AttachedToCS=CS1  CG=Right$CG$[-20.2 12.5544 48.3902]$WORLD$WORLD$mm$[0 0 1;0.442295 -0.89687 0;0.89687 0.442295 0]$3x3 Transform$rad$WORLD$false$113::CG(AUTOGEN)  WorkingFrames=Right$CS1$[-20.2 12.5544 48.3902]$WORLD$WORLD$mm$[0 0 1;0.442295 -0.89687 0;0.89687 0.442295 0]$3x3 Transform$rad$WORLD$false$113::CS1(AUTOGEN)#Left$CS2$[-25.1002 3.26616 29.556]$WORLD$WORLD$mm$[1 0 0;0 1 0;0 0 1]$3x3 Transform$rad$WORLD$true$113:-:74::113(AUTOGEN)#Right$CS3$[-25.1 21.8426 67.2245]$WORLD$WORLD$mm$[1 0 0;0 1 0;0 0 1]$3x3 Transform$rad$WORLD$true$110:-:113::113(AUTOGEN)  CGPos=[-20.2 12.5544 48.3902]  CGRot=[0 0 1;0.442295 -0.89687 0;0.89687 0.442295 0]  CS0Pos=[]  CS0Rot=[]  CS1Pos=[-20.2 12.5544 48.3902]  CS1Rot=[0 0 1;0.442295 -0.89687 0;0.89687 0.442295 0]  CS2Pos=[-25.1002 3.26616 29.556]  CS2Rot=[1 0 0;0 1 0;0 0 1]  CS3Pos=[-25.1 21.8426 67.2245]  CS3Rot=[1 0 0;0 1 0;0 0 1]  CS4Pos=[]  CS4Rot=[]  CS5Pos=[]  CS5Rot=[]  CS6Pos=[]  CS6Rot=[]  CS7Pos=[]  CS7Rot=[]  CS8Pos=[]  CS8Rot=[]  CS9Pos=[]  CS9Rot=[]  CS10Pos=[]  CS10Rot=[]  CS11Pos=[]  CS11Rot=[]  CS12Pos=[]  CS12Rot=[]  CS13Pos=[]  CS13Rot=[]  CS14Pos=[]  CS14Rot=[]  CS15Pos=[]  CS15Rot=[]  CS16Pos=[]  CS16Rot=[]  CS17Pos=[]  CS17Rot=[]  CS18Pos=[]  CS18Rot=[]  CS19Pos=[]  CS19Rot=[]  CS20Pos=[]  CS20Rot=[]
  PLEUEL-3 : mblibv1/Bodies/Body  DialogController=MECH.DynMechDlgSource  PhysicalDomain=mechanical  SubClassName=Unknown  LeftPortType=workingframe  RightPortType=workingframe  LConnTagsString=CS2  RConnTagsString=CS3  PMImportedID=104  UpdateFromCAD=on  DialogClass=MechanicalBodyBlock  Mass=4.9128e+006  MassUnits=kg  InertiaUnits=kg*m^2  Inertia=[14.226,0,0;0,458.442,0;0,0,380.048]  Shape=Cylinder  ShapeDims=[1 1]  ShapeUnits=m  ShapeUse=false  Density=1  DensityUnits=kg/m^3  DensityUse=false  GraphicsMode=GFXFILE  GraphicsFileName=PLEUEL_prt.stl  BodyColorSelMode=MACHINE_DEFAULT  BodyColor=[1 0 0]  AttachedToCS=CS1  CG=Right$CG$[-20.2 37.3067 5.22453]$WORLD$WORLD$mm$[0 0 1;0.968558 0.248787 0;-0.248787 0.968558 0]$3x3 Transform$rad$WORLD$false$104::CG(AUTOGEN)  WorkingFrames=Right$CS1$[-20.2 37.3067 5.22453]$WORLD$WORLD$mm$[0 0 1;0.968558 0.248787 0;-0.248787 0.968558 0]$3x3 Transform$rad$WORLD$false$104::CS1(AUTOGEN)#Left$CS2$[-29 16.9669 10.4491]$WORLD$WORLD$mm$[1 0 0;0 1 0;0 0 1]$3x3 Transform$rad$WORLD$true$104:-:74::104(AUTOGEN)#Right$CS3$[-25.1 57.6465 0]$WORLD$WORLD$mm$[1 0 0;0 1 0;0 0 1]$3x3 Transform$rad$WORLD$true$104:-:73::104(AUTOGEN)  CGPos=[-20.2 37.3067 5.22453]  CGRot=[0 0 1;0.968558 0.248787 0;-0.248787 0.968558 0]  CS0Pos=[]  CS0Rot=[]  CS1Pos=[-20.2 37.3067 5.22453]  CS1Rot=[0 0 1;0.968558 0.248787 0;-0.248787 0.968558 0]  CS2Pos=[-29 16.9669 10.4491]  CS2Rot=[1 0 0;0 1 0;0 0 1]  CS3Pos=[-25.1 57.6465 0]  CS3Rot=[1 0 0;0 1 0;0 0 1]  CS4Pos=[]  CS4Rot=[]  CS5Pos=[]  CS5Rot=[]  CS6Pos=[]  CS6Rot=[]  CS7Pos=[]  CS7Rot=[]  CS8Pos=[]  CS8Rot=[]  CS9Pos=[]  CS9Rot=[]  CS10Pos=[]  CS10Rot=[]  CS11Pos=[]  CS11Rot=[]  CS12Pos=[]  CS12Rot=[]  CS13Pos=[]  CS13Rot=[]  CS14Pos=[]  CS14Rot=[]  CS15Pos=[]  CS15Rot=[]  CS16Pos=[]  CS16Rot=[]  CS17Pos=[]  CS17Rot=[]  CS18Pos=[]  CS18Rot=[]  CS19Pos=[]  CS19Rot=[]  CS20Pos=[]  CS20Rot=[]
  PROPELLER : mblibv1/Bodies/Body  DialogController=MECH.DynMechDlgSource  PhysicalDomain=mechanical  SubClassName=Unknown  LeftPortType=workingframe  RightPortType=workingframe  LConnTagsString=CS2  RConnTagsString=CS3|CS4  PMImportedID=111  UpdateFromCAD=on  DialogClass=MechanicalBodyBlock  Mass=3.09e+007  MassUnits=kg  InertiaUnits=kg*m^2  Inertia=[5969.93,-2644.36,0;-2644.36,31773.2,0;0,0,31794]  Shape=Cylinder  ShapeDims=[1 1]  ShapeUnits=m  ShapeUse=false  Density=1  DensityUnits=kg/m^3  DensityUse=false  GraphicsMode=CONVHULL  GraphicsFileName=PROPELLER3_prt.stl  BodyColorSelMode=COLORPALETTE  BodyColor=[0.16863 0.50588 0.33725]  AttachedToCS=CS1  CG=Right$CG$[65.5473 -42.515 -5.01496]$WORLD$WORLD$mm$[0 -1 0;-0.275687 0 -0.961247;0.961247 0 -0.275687]$3x3 Transform$rad$WORLD$false$111::CG(AUTOGEN)  WorkingFrames=Right$CS1$[65.5473 -42.515 -5.01496]$WORLD$WORLD$mm$[0 -1 0;-0.275687 0 -0.961247;0.961247 0 -0.275687]$3x3 Transform$rad$WORLD$false$111::CS1(AUTOGEN)#Left$CS2$[90.95 0 0]$WORLD$WORLD$mm$[1 0 0;0 1 0;0 0 1]$3x3 Transform$rad$WORLD$true$111:-:76::111(AUTOGEN)#Right$CS3$[77.2473 0 0]$WORLD$WORLD$mm$[1 0 0;0 1 0;0 0 1]$3x3 Transform$rad$WORLD$true$111:-:112::111(AUTOGEN)#Right$CS4$[0 0 0]$CS3$CS3$mm$[1 0 0;0 1 0;0 0 1]$3x3 Transform$rad$WORLD$true$none  CGPos=[65.5473 -42.515 -5.01496]  CGRot=[0 -1 0;-0.275687 0 -0.961247;0.961247 0 -0.275687]  CS0Pos=[]  CS0Rot=[]  CS1Pos=[65.5473 -42.515 -5.01496]  CS1Rot=[0 -1 0;-0.275687 0 -0.961247;0.961247 0 -0.275687]  CS2Pos=[90.95 0 0]  CS2Rot=[1 0 0;0 1 0;0 0 1]  CS3Pos=[77.2473 0 0]  CS3Rot=[1 0 0;0 1 0;0 0 1]  CS4Pos=[0 0 0]  CS4Rot=[1 0 0;0 1 0;0 0 1]  CS5Pos=[]  CS5Rot=[]  CS6Pos=[]  CS6Rot=[]  CS7Pos=[]  CS7Rot=[]  CS8Pos=[]  CS8Rot=[]  CS9Pos=[]  CS9Rot=[]  CS10Pos=[]  CS10Rot=[]  CS11Pos=[]  CS11Rot=[]  CS12Pos=[]  CS12Rot=[]  CS13Pos=[]  CS13Rot=[]  CS14Pos=[]  CS14Rot=[]  CS15Pos=[]  CS15Rot=[]  CS16Pos=[]  CS16Rot=[]  CS17Pos=[]  CS17Rot=[]  CS18Pos=[]  CS18Rot=[]  CS19Pos=[]  CS19Rot=[]  CS20Pos=[]  CS20Rot=[]
  Revolute : mblibv1/Joints/Revolute  DialogController=MECH.DynMechDlgSource  PhysicalDomain=mechanical  SubClassName=Unknown  LeftPortType=blob  RightPortType=blob  LConnTagsString=__newl0  RConnTagsString=__newr0  PMImportedID=:-:RootPart  UpdateFromCAD=on  NumSAPorts=0  CutJoint=off  MarkAsCut=off  Primitives=prismatic  PrimitiveProps=R1$WORLD$[-1,0,0]$revolute  DialogClass=JointBlock  R1Axis=[-1,0,0]
  Revolute1 : mblibv1/Joints/Revolute  DialogController=MECH.DynMechDlgSource  PhysicalDomain=mechanical  SubClassName=Unknown  LeftPortType=blob  RightPortType=blob  LConnTagsString=__newl0  RConnTagsString=__newr0  PMImportedID=74:-:79  UpdateFromCAD=on  NumSAPorts=0  CutJoint=off  MarkAsCut=off  Primitives=prismatic  PrimitiveProps=R1$WORLD$[1,0,0]$revolute  DialogClass=JointBlock  R1Axis=[1,0,0]
  Revolute2 : mblibv1/Joints/Revolute  DialogController=MECH.DynMechDlgSource  PhysicalDomain=mechanical  SubClassName=Unknown  LeftPortType=blob  RightPortType=blob  LConnTagsString=__newl0  RConnTagsString=__newr0  PMImportedID=108:-:74  UpdateFromCAD=on  NumSAPorts=0  CutJoint=off  MarkAsCut=off  Primitives=prismatic  PrimitiveProps=R1$WORLD$[1,0,0]$revolute  DialogClass=JointBlock  R1Axis=[1,0,0]
  Revolute3 : mblibv1/Joints/Revolute  DialogController=MECH.DynMechDlgSource  PhysicalDomain=mechanical  SubClassName=Unknown  LeftPortType=blob  RightPortType=blob  LConnTagsString=__newl0  RConnTagsString=__newr0  PMImportedID=113:-:74  UpdateFromCAD=on  NumSAPorts=0  CutJoint=off  MarkAsCut=off  Primitives=prismatic  PrimitiveProps=R1$WORLD$[1,0,0]$revolute  DialogClass=JointBlock  R1Axis=[1,0,0]
  Revolute4 : mblibv1/Joints/Revolute  DialogController=MECH.DynMechDlgSource  PhysicalDomain=mechanical  SubClassName=Unknown  LeftPortType=blob  RightPortType=blob  LConnTagsString=__newl0  RConnTagsString=__newr0  PMImportedID=104:-:74  UpdateFromCAD=on  NumSAPorts=0  CutJoint=off  MarkAsCut=off  Primitives=prismatic  PrimitiveProps=R1$WORLD$[1,0,0]$revolute  DialogClass=JointBlock  R1Axis=[1,0,0]
  RootGround : mblibv1/Bodies/Ground  DialogController=MECH.DynMechDlgSource  SystemSampleTime=-1  PMImportedID=RootGround  UpdateFromCAD=on  LeftPortType=env  RightPortType=workingframe  PhysicalDomain=Mechanical  DialogClass=GroundBlock  CoordPosition=[-14.614,-0.00495788,0.187193]  CoordPositionUnits=mm  StateVectorMgrId=1  MachineId=[2 1]  ShowEnvPort=on
  RootPart : mblibv1/Bodies/Body  DialogController=MECH.DynMechDlgSource  PhysicalDomain=mechanical  SubClassName=Unknown  LeftPortType=workingframe  RightPortType=workingframe  LConnTagsString=CS18  RConnTagsString=CS2|CS3|CS4|CS5|CS6|CS7|CS8|CS9|CS10|CS11|CS12|CS13|CS14|CS15|CS16|CS17  PMImportedID=RootPart  UpdateFromCAD=on  DialogClass=MechanicalBodyBlock  Mass=0  MassUnits=kg  InertiaUnits=kg*m^2  Inertia=[0,0,0;0,0,0;0,0,0]  Shape=Cylinder  ShapeDims=[1 1]  ShapeUnits=m  ShapeUse=false  Density=1  DensityUnits=kg/m^3  DensityUse=false  GraphicsMode=MACHINE_DEFAULT  BodyColorSelMode=MACHINE_DEFAULT  BodyColor=[1 0 0]  AttachedToCS=CS1  CG=Right$CG$[-14.614 -0.00495788 0.187193]$WORLD$WORLD$mm$[1 0 0;0 1 0;0 0 1]$3x3 Transform$rad$WORLD$false$RootPart::CG(AUTOGEN)  WorkingFrames=Right$CS1$[0 0 0]$WORLD$WORLD$mm$[1 0 0;0 1 0;0 0 1]$3x3 Transform$rad$WORLD$false$RootPart::CS1(AUTOGEN)#Right$CS2$[-25 -66.7188 -48.4741]$WORLD$WORLD$mm$[1 0 0;0 1 0;0 0 1]$3x3 Transform$rad$WORLD$true$44:-:RootPart::RootPart(AUTOGEN)#Right$CS3$[-25 -66.7188 48.4741]$WORLD$WORLD$mm$[1 0 0;0 1 0;0 0 1]$3x3 Transform$rad$WORLD$true$91:-:RootPart::RootPart(AUTOGEN)#Right$CS4$[-25 82.469 0]$WORLD$WORLD$mm$[1 0 0;0 1 0;0 0 1]$3x3 Transform$rad$WORLD$true$20:-:RootPart::RootPart(AUTOGEN)#Right$CS5$[-25 25.4843 -78.4327]$WORLD$WORLD$mm$[1 0 0;0 1 0;0 0 1]$3x3 Transform$rad$WORLD$true$31:-:RootPart::RootPart(AUTOGEN)#Right$CS6$[-25 25.4843 78.4327]$WORLD$WORLD$mm$[1 0 0;0 1 0;0 0 1]$3x3 Transform$rad$WORLD$true$64:-:RootPart::RootPart(AUTOGEN)#Right$CS7$[-25 -37.6193 -27.332]$WORLD$WORLD$mm$[1 0 0;0 1 0;0 0 1]$3x3 Transform$rad$WORLD$true$43:-:RootPart::RootPart(AUTOGEN)#Right$CS8$[-25 46.5 0]$WORLD$WORLD$mm$[1 0 0;0 1 0;0 0 1]$3x3 Transform$rad$WORLD$true$19:-:RootPart::RootPart(AUTOGEN)#Right$CS9$[-25 14.3693 -44.2241]$WORLD$WORLD$mm$[1 0 0;0 1 0;0 0 1]$3x3 Transform$rad$WORLD$true$30:-:RootPart::RootPart(AUTOGEN)#Right$CS10$[-25 14.3693 44.2241]$WORLD$WORLD$mm$[1 0 0;0 1 0;0 0 1]$3x3 Transform$rad$WORLD$true$63:-:RootPart::RootPart(AUTOGEN)#Right$CS11$[-25 -37.6193 27.332]$WORLD$WORLD$mm$[1 0 0;0 1 0;0 0 1]$3x3 Transform$rad$WORLD$true$90:-:RootPart::RootPart(AUTOGEN)#Right$CS12$[-25 -51.4707 -37.3957]$WORLD$WORLD$mm$[1 0 0;0 1 0;0 0 1]$3x3 Transform$rad$WORLD$true$42:-:RootPart::RootPart(AUTOGEN)#Right$CS13$[-25 63.6213 0]$WORLD$WORLD$mm$[1 0 0;0 1 0;0 0 1]$3x3 Transform$rad$WORLD$true$18:-:RootPart::RootPart(AUTOGEN)#Right$CS14$[-25 19.6601 -60.5075]$WORLD$WORLD$mm$[1 0 0;0 1 0;0 0 1]$3x3 Transform$rad$WORLD$true$29:-:RootPart::RootPart(AUTOGEN)#Right$CS15$[-25 19.6601 60.5075]$WORLD$WORLD$mm$[1 0 0;0 1 0;0 0 1]$3x3 Transform$rad$WORLD$true$62:-:RootPart::RootPart(AUTOGEN)#Right$CS16$[-25 -51.4707 37.3957]$WORLD$WORLD$mm$[1 0 0;0 1 0;0 0 1]$3x3 Transform$rad$WORLD$true$89:-:RootPart::RootPart(AUTOGEN)#Right$CS17$[-5.05 0 0]$WORLD$WORLD$mm$[1 0 0;0 1 0;0 0 1]$3x3 Transform$rad$WORLD$true$:-:RootPart::RootPart(AUTOGEN)#Left$CS18$[-14.614 -0.00495788 0.187193]$WORLD$WORLD$mm$[1 0 0;0 1 0;0 0 1]$3x3 Transform$rad$WORLD$true$RootGround:-:RootPart::RootPart(AUTOGEN)  CGPos=[-14.614 -0.00495788 0.187193]  CGRot=[1 0 0;0 1 0;0 0 1]  CS0Pos=[]  CS0Rot=[]  CS1Pos=[0 0 0]  CS1Rot=[1 0 0;0 1 0;0 0 1]  CS2Pos=[-25 -66.7188 -48.4741]  CS2Rot=[1 0 0;0 1 0;0 0 1]  CS3Pos=[-25 -66.7188 48.4741]  CS3Rot=[1 0 0;0 1 0;0 0 1]  CS4Pos=[-25 82.469 0]  CS4Rot=[1 0 0;0 1 0;0 0 1]  CS5Pos=[-25 25.4843 -78.4327]  CS5Rot=[1 0 0;0 1 0;0 0 1]  CS6Pos=[-25 25.4843 78.4327]  CS6Rot=[1 0 0;0 1 0;0 0 1]  CS7Pos=[-25 -37.6193 -27.332]  CS7Rot=[1 0 0;0 1 0;0 0 1]  CS8Pos=[-25 46.5 0]  CS8Rot=[1 0 0;0 1 0;0 0 1]  CS9Pos=[-25 14.3693 -44.2241]  CS9Rot=[1 0 0;0 1 0;0 0 1]  CS10Pos=[-25 14.3693 44.2241]  CS10Rot=[1 0 0;0 1 0;0 0 1]  CS11Pos=[-25 -37.6193 27.332]  CS11Rot=[1 0 0;0 1 0;0 0 1]  CS12Pos=[-25 -51.4707 -37.3957]  CS12Rot=[1 0 0;0 1 0;0 0 1]  CS13Pos=[-25 63.6213 0]  CS13Rot=[1 0 0;0 1 0;0 0 1]  CS14Pos=[-25 19.6601 -60.5075]  CS14Rot=[1 0 0;0 1 0;0 0 1]  CS15Pos=[-25 19.6601 60.5075]  CS15Rot=[1 0 0;0 1 0;0 0 1]  CS16Pos=[-25 -51.4707 37.3957]  CS16Rot=[1 0 0;0 1 0;0 0 1]  CS17Pos=[-5.05 0 0]  CS17Rot=[1 0 0;0 1 0;0 0 1]  CS18Pos=[-14.614 -0.00495788 0.187193]  CS18Rot=[1 0 0;0 1 0;0 0 1]  CS19Pos=[]  CS19Rot=[]  CS20Pos=[]  CS20Rot=[]
  SPINNER : mblibv1/Bodies/Body  DialogController=MECH.DynMechDlgSource  PhysicalDomain=mechanical  SubClassName=Unknown  LeftPortType=workingframe  RightPortType=workingframe  LConnTagsString=CS2  PMImportedID=112  UpdateFromCAD=on  DialogClass=MechanicalBodyBlock  Mass=0  MassUnits=kg  InertiaUnits=kg*m^2  Inertia=[0,0,0;0,0,0;0,0,0]  Shape=Cylinder  ShapeDims=[1 1]  ShapeUnits=m  ShapeUse=false  Density=1  DensityUnits=kg/m^3  DensityUse=false  GraphicsMode=GFXFILE  GraphicsFileName=SPINNER_prt.stl  BodyColorSelMode=MACHINE_DEFAULT  BodyColor=[1 0 0]  AttachedToCS=CS1  CG=Right$CG$[77.2473 0 0]$WORLD$WORLD$mm$[1 0 0;0 -0.961247 0.275687;0 -0.275687 -0.961247]$3x3 Transform$rad$WORLD$false$112::CG(AUTOGEN)  WorkingFrames=Right$CS1$[77.2473 0 0]$WORLD$WORLD$mm$[1 0 0;0 -0.961247 0.275687;0 -0.275687 -0.961247]$3x3 Transform$rad$WORLD$false$112::CS1(AUTOGEN)#Left$CS2$[77.2473 0 0]$WORLD$WORLD$mm$[1 0 0;0 1 0;0 0 1]$3x3 Transform$rad$WORLD$true$111:-:112::112(AUTOGEN)  CGPos=[77.2473 0 0]  CGRot=[1 0 0;0 -0.961247 0.275687;0 -0.275687 -0.961247]  CS0Pos=[]  CS0Rot=[]  CS1Pos=[77.2473 0 0]  CS1Rot=[1 0 0;0 -0.961247 0.275687;0 -0.275687 -0.961247]  CS2Pos=[77.2473 0 0]  CS2Rot=[1 0 0;0 1 0;0 0 1]  CS3Pos=[]  CS3Rot=[]  CS4Pos=[]  CS4Rot=[]  CS5Pos=[]  CS5Rot=[]  CS6Pos=[]  CS6Rot=[]  CS7Pos=[]  CS7Rot=[]  CS8Pos=[]  CS8Rot=[]  CS9Pos=[]  CS9Rot=[]  CS10Pos=[]  CS10Rot=[]  CS11Pos=[]  CS11Rot=[]  CS12Pos=[]  CS12Rot=[]  CS13Pos=[]  CS13Rot=[]  CS14Pos=[]  CS14Rot=[]  CS15Pos=[]  CS15Rot=[]  CS16Pos=[]  CS16Rot=[]  CS17Pos=[]  CS17Rot=[]  CS18Pos=[]  CS18Rot=[]  CS19Pos=[]  CS19Rot=[]  CS20Pos=[]  CS20Rot=[]
  Scope : Scope
      settings: YMin=-1  YMax=1
  Weld : mblibv1/Joints/Weld  DialogController=MECH.DynMechDlgSource  PhysicalDomain=mechanical  SubClassName=Unknown  LeftPortType=blob  RightPortType=blob  LConnTagsString=__newl0  RConnTagsString=__newr0  PMImportedID=44:-:RootPart  UpdateFromCAD=on  NumSAPorts=0  CutJoint=off  MarkAsCut=off  Primitives=weld  PrimitiveProps=W$WORLD$[0.57735,0.57735,0.57735]$weld  DialogClass=JointBlock  WAxis=[0.57735,0.57735,0.57735]
  Weld1 : mblibv1/Joints/Weld  DialogController=MECH.DynMechDlgSource  PhysicalDomain=mechanical  SubClassName=Unknown  LeftPortType=blob  RightPortType=blob  LConnTagsString=__newl0  RConnTagsString=__newr0  PMImportedID=91:-:RootPart  UpdateFromCAD=on  NumSAPorts=0  CutJoint=off  MarkAsCut=off  Primitives=weld  PrimitiveProps=W$WORLD$[0.57735,0.57735,0.57735]$weld  DialogClass=JointBlock  WAxis=[0.57735,0.57735,0.57735]
  Weld10 : mblibv1/Joints/Weld  DialogController=MECH.DynMechDlgSource  PhysicalDomain=mechanical  SubClassName=Unknown  LeftPortType=blob  RightPortType=blob  LConnTagsString=__newl0  RConnTagsString=__newr0  PMImportedID=42:-:RootPart  UpdateFromCAD=on  NumSAPorts=0  CutJoint=off  MarkAsCut=off  Primitives=weld  PrimitiveProps=W$WORLD$[0.57735,0.57735,0.57735]$weld  DialogClass=JointBlock  WAxis=[0.57735,0.57735,0.57735]
  Weld11 : mblibv1/Joints/Weld  DialogController=MECH.DynMechDlgSource  PhysicalDomain=mechanical  SubClassName=Unknown  LeftPortType=blob  RightPortType=blob  LConnTagsString=__newl0  RConnTagsString=__newr0  PMImportedID=18:-:RootPart  UpdateFromCAD=on  NumSAPorts=0  CutJoint=off  MarkAsCut=off  Primitives=weld  PrimitiveProps=W$WORLD$[0.57735,0.57735,0.57735]$weld  DialogClass=JointBlock  WAxis=[0.57735,0.57735,0.57735]
  Weld12 : mblibv1/Joints/Weld  DialogController=MECH.DynMechDlgSource  PhysicalDomain=mechanical  SubClassName=Unknown  LeftPortType=blob  RightPortType=blob  LConnTagsString=__newl0  RConnTagsString=__newr0  PMImportedID=29:-:RootPart  UpdateFromCAD=on  NumSAPorts=0  CutJoint=off  MarkAsCut=off  Primitives=weld  PrimitiveProps=W$WORLD$[0.57735,0.57735,0.57735]$weld  DialogClass=JointBlock  WAxis=[0.57735,0.57735,0.57735]
  Weld13 : mblibv1/Joints/Weld  DialogController=MECH.DynMechDlgSource  PhysicalDomain=mechanical  SubClassName=Unknown  LeftPortType=blob  RightPortType=blob  LConnTagsString=__newl0  RConnTagsString=__newr0  PMImportedID=62:-:RootPart  UpdateFromCAD=on  NumSAPorts=0  CutJoint=off  MarkAsCut=off  Primitives=weld  PrimitiveProps=W$WORLD$[0.57735,0.57735,0.57735]$weld  DialogClass=JointBlock  WAxis=[0.57735,0.57735,0.57735]
  Weld14 : mblibv1/Joints/Weld  DialogController=MECH.DynMechDlgSource  PhysicalDomain=mechanical  SubClassName=Unknown  LeftPortType=blob  RightPortType=blob  LConnTagsString=__newl0  RConnTagsString=__newr0  PMImportedID=89:-:RootPart  UpdateFromCAD=on  NumSAPorts=0  CutJoint=off  MarkAsCut=off  Primitives=weld  PrimitiveProps=W$WORLD$[0.57735,0.57735,0.57735]$weld  DialogClass=JointBlock  WAxis=[0.57735,0.57735,0.57735]
  Weld15 : mblibv1/Joints/Weld  DialogController=MECH.DynMechDlgSource  PhysicalDomain=mechanical  SubClassName=Unknown  LeftPortType=blob  RightPortType=blob  LConnTagsString=__newl0  RConnTagsString=__newr0  PMImportedID=111:-:76  UpdateFromCAD=on  NumSAPorts=0  CutJoint=off  MarkAsCut=off  Primitives=weld  PrimitiveProps=W$WORLD$[0.57735,0.57735,0.57735]$weld  DialogClass=JointBlock  WAxis=[0.57735,0.57735,0.57735]
  Weld16 : mblibv1/Joints/Weld  DialogController=MECH.DynMechDlgSource  PhysicalDomain=mechanical  SubClassName=Unknown  LeftPortType=blob  RightPortType=blob  LConnTagsString=__newl0  RConnTagsString=__newr0  PMImportedID=111:-:112  UpdateFromCAD=on  NumSAPorts=0  CutJoint=off  MarkAsCut=off  Primitives=weld  PrimitiveProps=W$WORLD$[0.57735,0.57735,0.57735]$weld  DialogClass=JointBlock  WAxis=[0.57735,0.57735,0.57735]
  Weld17 : mblibv1/Joints/Weld  DialogController=MECH.DynMechDlgSource  PhysicalDomain=mechanical  SubClassName=Unknown  LeftPortType=blob  RightPortType=blob  LConnTagsString=__newl0  RConnTagsString=__newr0  PMImportedID=RootGround:-:RootPart  UpdateFromCAD=on  NumSAPorts=0  CutJoint=off  MarkAsCut=off  Primitives=weld  PrimitiveProps=W$WORLD$[0.57735,0.57735,0.57735]$weld  DialogClass=JointBlock  WAxis=[0.57735,0.57735,0.57735]
  Weld2 : mblibv1/Joints/Weld  DialogController=MECH.DynMechDlgSource  PhysicalDomain=mechanical  SubClassName=Unknown  LeftPortType=blob  RightPortType=blob  LConnTagsString=__newl0  RConnTagsString=__newr0  PMImportedID=20:-:RootPart  UpdateFromCAD=on  NumSAPorts=0  CutJoint=off  MarkAsCut=off  Primitives=weld  PrimitiveProps=W$WORLD$[0.57735,0.57735,0.57735]$weld  DialogClass=JointBlock  WAxis=[0.57735,0.57735,0.57735]
  Weld3 : mblibv1/Joints/Weld  DialogController=MECH.DynMechDlgSource  PhysicalDomain=mechanical  SubClassName=Unknown  LeftPortType=blob  RightPortType=blob  LConnTagsString=__newl0  RConnTagsString=__newr0  PMImportedID=31:-:RootPart  UpdateFromCAD=on  NumSAPorts=0  CutJoint=off  MarkAsCut=off  Primitives=weld  PrimitiveProps=W$WORLD$[0.57735,0.57735,0.57735]$weld  DialogClass=JointBlock  WAxis=[0.57735,0.57735,0.57735]
  Weld4 : mblibv1/Joints/Weld  DialogController=MECH.DynMechDlgSource  PhysicalDomain=mechanical  SubClassName=Unknown  LeftPortType=blob  RightPortType=blob  LConnTagsString=__newl0  RConnTagsString=__newr0  PMImportedID=64:-:RootPart  UpdateFromCAD=on  NumSAPorts=0  CutJoint=off  MarkAsCut=off  Primitives=weld  PrimitiveProps=W$WORLD$[0.57735,0.57735,0.57735]$weld  DialogClass=JointBlock  WAxis=[0.57735,0.57735,0.57735]
  Weld5 : mblibv1/Joints/Weld  DialogController=MECH.DynMechDlgSource  PhysicalDomain=mechanical  SubClassName=Unknown  LeftPortType=blob  RightPortType=blob  LConnTagsString=__newl0  RConnTagsString=__newr0  PMImportedID=43:-:RootPart  UpdateFromCAD=on  NumSAPorts=0  CutJoint=off  MarkAsCut=off  Primitives=weld  PrimitiveProps=W$WORLD$[0.57735,0.57735,0.57735]$weld  DialogClass=JointBlock  WAxis=[0.57735,0.57735,0.57735]
  Weld6 : mblibv1/Joints/Weld  DialogController=MECH.DynMechDlgSource  PhysicalDomain=mechanical  SubClassName=Unknown  LeftPortType=blob  RightPortType=blob  LConnTagsString=__newl0  RConnTagsString=__newr0  PMImportedID=19:-:RootPart  UpdateFromCAD=on  NumSAPorts=0  CutJoint=off  MarkAsCut=off  Primitives=weld  PrimitiveProps=W$WORLD$[0.57735,0.57735,0.57735]$weld  DialogClass=JointBlock  WAxis=[0.57735,0.57735,0.57735]
  Weld7 : mblibv1/Joints/Weld  DialogController=MECH.DynMechDlgSource  PhysicalDomain=mechanical  SubClassName=Unknown  LeftPortType=blob  RightPortType=blob  LConnTagsString=__newl0  RConnTagsString=__newr0  PMImportedID=30:-:RootPart  UpdateFromCAD=on  NumSAPorts=0  CutJoint=off  MarkAsCut=off  Primitives=weld  PrimitiveProps=W$WORLD$[0.57735,0.57735,0.57735]$weld  DialogClass=JointBlock  WAxis=[0.57735,0.57735,0.57735]
  Weld8 : mblibv1/Joints/Weld  DialogController=MECH.DynMechDlgSource  PhysicalDomain=mechanical  SubClassName=Unknown  LeftPortType=blob  RightPortType=blob  LConnTagsString=__newl0  RConnTagsString=__newr0  PMImportedID=63:-:RootPart  UpdateFromCAD=on  NumSAPorts=0  CutJoint=off  MarkAsCut=off  Primitives=weld  PrimitiveProps=W$WORLD$[0.57735,0.57735,0.57735]$weld  DialogClass=JointBlock  WAxis=[0.57735,0.57735,0.57735]
  Weld9 : mblibv1/Joints/Weld  DialogController=MECH.DynMechDlgSource  PhysicalDomain=mechanical  SubClassName=Unknown  LeftPortType=blob  RightPortType=blob  LConnTagsString=__newl0  RConnTagsString=__newr0  PMImportedID=90:-:RootPart  UpdateFromCAD=on  NumSAPorts=0  CutJoint=off  MarkAsCut=off  Primitives=weld  PrimitiveProps=W$WORLD$[0.57735,0.57735,0.57735]$weld  DialogClass=JointBlock  WAxis=[0.57735,0.57735,0.57735]
  ZYL-KOPF : mblibv1/Bodies/Body  DialogController=MECH.DynMechDlgSource  PhysicalDomain=mechanical  SubClassName=Unknown  LeftPortType=workingframe  RightPortType=workingframe  LConnTagsString=CS2  PMImportedID=44  UpdateFromCAD=on  DialogClass=MechanicalBodyBlock  Mass=0  MassUnits=kg  InertiaUnits=kg*m^2  Inertia=eye(3)  Shape=Cylinder  ShapeDims=[1 1]  ShapeUnits=m  ShapeUse=false  Density=1  DensityUnits=kg/m^3  DensityUse=false  GraphicsMode=CONVHULL  GraphicsFileName=ZYL-KOPF_prt.stl  BodyColorSelMode=MACHINE_DEFAULT  BodyColor=[1 0 0]  AttachedToCS=CS1  CG=Right$CG$[-25 -66.7188 -48.4741]$WORLD$WORLD$mm$[0 0 1;-0.587785 -0.809017 0;0.809017 -0.587785 0]$3x3 Transform$rad$WORLD$false$44::CG(AUTOGEN)  WorkingFrames=Right$CS1$[-25 -66.7188 -48.4741]$WORLD$WORLD$mm$[0 0 1;-0.587785 -0.809017 0;0.809017 -0.587785 0]$3x3 Transform$rad$WORLD$false$44::CS1(AUTOGEN)#Left$CS2$[-25 -66.7188 -48.4741]$WORLD$WORLD$mm$[1 0 0;0 1 0;0 0 1]$3x3 Transform$rad$WORLD$true$44:-:RootPart::44(AUTOGEN)  CGPos=[-25 -66.7188 -48.4741]  CGRot=[0 0 1;-0.587785 -0.809017 0;0.809017 -0.587785 0]  CS0Pos=[]  CS0Rot=[]  CS1Pos=[-25 -66.7188 -48.4741]  CS1Rot=[0 0 1;-0.587785 -0.809017 0;0.809017 -0.587785 0]  CS2Pos=[-25 -66.7188 -48.4741]  CS2Rot=[1 0 0;0 1 0;0 0 1]  CS3Pos=[]  CS3Rot=[]  CS4Pos=[]  CS4Rot=[]  CS5Pos=[]  CS5Rot=[]  CS6Pos=[]  CS6Rot=[]  CS7Pos=[]  CS7Rot=[]  CS8Pos=[]  CS8Rot=[]  CS9Pos=[]  CS9Rot=[]  CS10Pos=[]  CS10Rot=[]  CS11Pos=[]  CS11Rot=[]  CS12Pos=[]  CS12Rot=[]  CS13Pos=[]  CS13Rot=[]  CS14Pos=[]  CS14Rot=[]  CS15Pos=[]  CS15Rot=[]  CS16Pos=[]  CS16Rot=[]  CS17Pos=[]  CS17Rot=[]  CS18Pos=[]  CS18Rot=[]  CS19Pos=[]  CS19Rot=[]  CS20Pos=[]  CS20Rot=[]
  ZYL-KOPF-1 : mblibv1/Bodies/Body  DialogController=MECH.DynMechDlgSource  PhysicalDomain=mechanical  SubClassName=Unknown  LeftPortType=workingframe  RightPortType=workingframe  LConnTagsString=CS2  PMImportedID=91  UpdateFromCAD=on  DialogClass=MechanicalBodyBlock  Mass=1  MassUnits=kg  InertiaUnits=kg*m^2  Inertia=eye(3)  Shape=Cylinder  ShapeDims=[1 1]  ShapeUnits=m  ShapeUse=false  Density=1  DensityUnits=kg/m^3  DensityUse=false  GraphicsMode=CONVHULL  GraphicsFileName=ZYL-KOPF_prt.stl  BodyColorSelMode=MACHINE_DEFAULT  BodyColor=[1 0 0]  AttachedToCS=CS1  CG=Right$CG$[-25 -66.7188 48.4741]$WORLD$WORLD$mm$[0 0 1;0.587785 -0.809017 0;0.809017 0.587785 0]$3x3 Transform$rad$WORLD$false$91::CG(AUTOGEN)  WorkingFrames=Right$CS1$[-25 -66.7188 48.4741]$WORLD$WORLD$mm$[0 0 1;0.587785 -0.809017 0;0.809017 0.587785 0]$3x3 Transform$rad$WORLD$false$91::CS1(AUTOGEN)#Left$CS2$[-25 -66.7188 48.4741]$WORLD$WORLD$mm$[1 0 0;0 1 0;0 0 1]$3x3 Transform$rad$WORLD$true$91:-:RootPart::91(AUTOGEN)  CGPos=[-25 -66.7188 48.4741]  CGRot=[0 0 1;0.587785 -0.809017 0;0.809017 0.587785 0]  CS0Pos=[]  CS0Rot=[]  CS1Pos=[-25 -66.7188 48.4741]  CS1Rot=[0 0 1;0.587785 -0.809017 0;0.809017 0.587785 0]  CS2Pos=[-25 -66.7188 48.4741]  CS2Rot=[1 0 0;0 1 0;0 0 1]  CS3Pos=[]  CS3Rot=[]  CS4Pos=[]  CS4Rot=[]  CS5Pos=[]  CS5Rot=[]  CS6Pos=[]  CS6Rot=[]  CS7Pos=[]  CS7Rot=[]  CS8Pos=[]  CS8Rot=[]  CS9Pos=[]  CS9Rot=[]  CS10Pos=[]  CS10Rot=[]  CS11Pos=[]  CS11Rot=[]  CS12Pos=[]  CS12Rot=[]  CS13Pos=[]  CS13Rot=[]  CS14Pos=[]  CS14Rot=[]  CS15Pos=[]  CS15Rot=[]  CS16Pos=[]  CS16Rot=[]  CS17Pos=[]  CS17Rot=[]  CS18Pos=[]  CS18Rot=[]  CS19Pos=[]  CS19Rot=[]  CS20Pos=[]  CS20Rot=[]
  ZYL-KOPF-2 : mblibv1/Bodies/Body  DialogController=MECH.DynMechDlgSource  PhysicalDomain=mechanical  SubClassName=Unknown  LeftPortType=workingframe  RightPortType=workingframe  LConnTagsString=CS2  PMImportedID=20  UpdateFromCAD=on  DialogClass=MechanicalBodyBlock  Mass=1  MassUnits=kg  InertiaUnits=kg*m^2  Inertia=eye(3)  Shape=Cylinder  ShapeDims=[1 1]  ShapeUnits=m  ShapeUse=false  Density=1  DensityUnits=kg/m^3  DensityUse=false  GraphicsMode=CONVHULL  GraphicsFileName=ZYL-KOPF_prt.stl  BodyColorSelMode=MACHINE_DEFAULT  BodyColor=[1 0 0]  AttachedToCS=CS1  CG=Right$CG$[-25 82.469 0]$WORLD$WORLD$mm$[0 0 1;0 1 0;-1 0 0]$3x3 Transform$rad$WORLD$false$20::CG(AUTOGEN)  WorkingFrames=Right$CS1$[-25 82.469 0]$WORLD$WORLD$mm$[0 0 1;0 1 0;-1 0 0]$3x3 Transform$rad$WORLD$false$20::CS1(AUTOGEN)#Left$CS2$[-25 82.469 0]$WORLD$WORLD$mm$[1 0 0;0 1 0;0 0 1]$3x3 Transform$rad$WORLD$true$20:-:RootPart::20(AUTOGEN)  CGPos=[-25 82.469 0]  CGRot=[0 0 1;0 1 0;-1 0 0]  CS0Pos=[]  CS0Rot=[]  CS1Pos=[-25 82.469 0]  CS1Rot=[0 0 1;0 1 0;-1 0 0]  CS2Pos=[-25 82.469 0]  CS2Rot=[1 0 0;0 1 0;0 0 1]  CS3Pos=[]  CS3Rot=[]  CS4Pos=[]  CS4Rot=[]  CS5Pos=[]  CS5Rot=[]  CS6Pos=[]  CS6Rot=[]  CS7Pos=[]  CS7Rot=[]  CS8Pos=[]  CS8Rot=[]  CS9Pos=[]  CS9Rot=[]  CS10Pos=[]  CS10Rot=[]  CS11Pos=[]  CS11Rot=[]  CS12Pos=[]  CS12Rot=[]  CS13Pos=[]  CS13Rot=[]  CS14Pos=[]  CS14Rot=[]  CS15Pos=[]  CS15Rot=[]  CS16Pos=[]  CS16Rot=[]  CS17Pos=[]  CS17Rot=[]  CS18Pos=[]  CS18Rot=[]  CS19Pos=[]  CS19Rot=[]  CS20Pos=[]  CS20Rot=[]
  ZYL-KOPF-3 : mblibv1/Bodies/Body  DialogController=MECH.DynMechDlgSource  PhysicalDomain=mechanical  SubClassName=Unknown  LeftPortType=workingframe  RightPortType=workingframe  LConnTagsString=CS2  PMImportedID=31  UpdateFromCAD=on  DialogClass=MechanicalBodyBlock  Mass=1  MassUnits=kg  InertiaUnits=kg*m^2  Inertia=eye(3)  Shape=Cylinder  ShapeDims=[1 1]  ShapeUnits=m  ShapeUse=false  Density=1  DensityUnits=kg/m^3  DensityUse=false  GraphicsMode=CONVHULL  GraphicsFileName=ZYL-KOPF_prt.stl  BodyColorSelMode=MACHINE_DEFAULT  BodyColor=[1 0 0]  AttachedToCS=CS1  CG=Right$CG$[-25 25.4843 -78.4327]$WORLD$WORLD$mm$[0 0 1;-0.951057 0.309017 0;-0.309017 -0.951057 0]$3x3 Transform$rad$WORLD$false$31::CG(AUTOGEN)  WorkingFrames=Right$CS1$[-25 25.4843 -78.4327]$WORLD$WORLD$mm$[0 0 1;-0.951057 0.309017 0;-0.309017 -0.951057 0]$3x3 Transform$rad$WORLD$false$31::CS1(AUTOGEN)#Left$CS2$[-25 25.4843 -78.4327]$WORLD$WORLD$mm$[1 0 0;0 1 0;0 0 1]$3x3 Transform$rad$WORLD$true$31:-:RootPart::31(AUTOGEN)  CGPos=[-25 25.4843 -78.4327]  CGRot=[0 0 1;-0.951057 0.309017 0;-0.309017 -0.951057 0]  CS0Pos=[]  CS0Rot=[]  CS1Pos=[-25 25.4843 -78.4327]  CS1Rot=[0 0 1;-0.951057 0.309017 0;-0.309017 -0.951057 0]  CS2Pos=[-25 25.4843 -78.4327]  CS2Rot=[1 0 0;0 1 0;0 0 1]  CS3Pos=[]  CS3Rot=[]  CS4Pos=[]  CS4Rot=[]  CS5Pos=[]  CS5Rot=[]  CS6Pos=[]  CS6Rot=[]  CS7Pos=[]  CS7Rot=[]  CS8Pos=[]  CS8Rot=[]  CS9Pos=[]  CS9Rot=[]  CS10Pos=[]  CS10Rot=[]  CS11Pos=[]  CS11Rot=[]  CS12Pos=[]  CS12Rot=[]  CS13Pos=[]  CS13Rot=[]  CS14Pos=[]  CS14Rot=[]  CS15Pos=[]  CS15Rot=[]  CS16Pos=[]  CS16Rot=[]  CS17Pos=[]  CS17Rot=[]  CS18Pos=[]  CS18Rot=[]  CS19Pos=[]  CS19Rot=[]  CS20Pos=[]  CS20Rot=[]
  ZYL-KOPF-4 : mblibv1/Bodies/Body  DialogController=MECH.DynMechDlgSource  PhysicalDomain=mechanical  SubClassName=Unknown  LeftPortType=workingframe  RightPortType=workingframe  LConnTagsString=CS2  PMImportedID=64  UpdateFromCAD=on  DialogClass=MechanicalBodyBlock  Mass=1  MassUnits=kg  InertiaUnits=kg*m^2  Inertia=eye(3)  Shape=Cylinder  ShapeDims=[1 1]  ShapeUnits=m  ShapeUse=false  Density=1  DensityUnits=kg/m^3  DensityUse=false  GraphicsMode=CONVHULL  GraphicsFileName=ZYL-KOPF_prt.stl  BodyColorSelMode=MACHINE_DEFAULT  BodyColor=[1 0 0]  AttachedToCS=CS1  CG=Right$CG$[-25 25.4843 78.4327]$WORLD$WORLD$mm$[0 0 1;0.951057 0.309017 0;-0.309017 0.951057 0]$3x3 Transform$rad$WORLD$false$64::CG(AUTOGEN)  WorkingFrames=Right$CS1$[-25 25.4843 78.4327]$WORLD$WORLD$mm$[0 0 1;0.951057 0.309017 0;-0.309017 0.951057 0]$3x3 Transform$rad$WORLD$false$64::CS1(AUTOGEN)#Left$CS2$[-25 25.4843 78.4327]$WORLD$WORLD$mm$[1 0 0;0 1 0;0 0 1]$3x3 Transform$rad$WORLD$true$64:-:RootPart::64(AUTOGEN)  CGPos=[-25 25.4843 78.4327]  CGRot=[0 0 1;0.951057 0.309017 0;-0.309017 0.951057 0]  CS0Pos=[]  CS0Rot=[]  CS1Pos=[-25 25.4843 78.4327]  CS1Rot=[0 0 1;0.951057 0.309017 0;-0.309017 0.951057 0]  CS2Pos=[-25 25.4843 78.4327]  CS2Rot=[1 0 0;0 1 0;0 0 1]  CS3Pos=[]  CS3Rot=[]  CS4Pos=[]  CS4Rot=[]  CS5Pos=[]  CS5Rot=[]  CS6Pos=[]  CS6Rot=[]  CS7Pos=[]  CS7Rot=[]  CS8Pos=[]  CS8Rot=[]  CS9Pos=[]  CS9Rot=[]  CS10Pos=[]  CS10Rot=[]  CS11Pos=[]  CS11Rot=[]  CS12Pos=[]  CS12Rot=[]  CS13Pos=[]  CS13Rot=[]  CS14Pos=[]  CS14Rot=[]  CS15Pos=[]  CS15Rot=[]  CS16Pos=[]  CS16Rot=[]  CS17Pos=[]  CS17Rot=[]  CS18Pos=[]  CS18Rot=[]  CS19Pos=[]  CS19Rot=[]  CS20Pos=[]  CS20Rot=[]
  ZYLINDER : mblibv1/Bodies/Body  DialogController=MECH.DynMechDlgSource  PhysicalDomain=mechanical  SubClassName=Unknown  LeftPortType=workingframe  RightPortType=workingframe  LConnTagsString=CS2  PMImportedID=43  UpdateFromCAD=on  DialogClass=MechanicalBodyBlock  Mass=0  MassUnits=kg  InertiaUnits=kg*m^2  Inertia=[0,0,0;0,0,0;0,0,0]  Shape=Cylinder  ShapeDims=[1 1]  ShapeUnits=m  ShapeUse=false  Density=1  DensityUnits=kg/m^3  DensityUse=false  GraphicsMode=GFXFILE  GraphicsFileName=ZYLINDER_prt.stl  BodyColorSelMode=MACHINE_DEFAULT  BodyColor=[1 0 0]  AttachedToCS=CS1  CG=Right$CG$[-25 -37.6193 -27.332]$WORLD$WORLD$mm$[0 0 1;-0.587785 -0.809017 0;0.809017 -0.587785 0]$3x3 Transform$rad$WORLD$false$43::CG(AUTOGEN)  WorkingFrames=Right$CS1$[-25 -37.6193 -27.332]$WORLD$WORLD$mm$[0 0 1;-0.587785 -0.809017 0;0.809017 -0.587785 0]$3x3 Transform$rad$WORLD$false$43::CS1(AUTOGEN)#Left$CS2$[-25 -37.6193 -27.332]$WORLD$WORLD$mm$[1 0 0;0 1 0;0 0 1]$3x3 Transform$rad$WORLD$true$43:-:RootPart::43(AUTOGEN)  CGPos=[-25 -37.6193 -27.332]  CGRot=[0 0 1;-0.587785 -0.809017 0;0.809017 -0.587785 0]  CS0Pos=[]  CS0Rot=[]  CS1Pos=[-25 -37.6193 -27.332]  CS1Rot=[0 0 1;-0.587785 -0.809017 0;0.809017 -0.587785 0]  CS2Pos=[-25 -37.6193 -27.332]  CS2Rot=[1 0 0;0 1 0;0 0 1]  CS3Pos=[]  CS3Rot=[]  CS4Pos=[]  CS4Rot=[]  CS5Pos=[]  CS5Rot=[]  CS6Pos=[]  CS6Rot=[]  CS7Pos=[]  CS7Rot=[]  CS8Pos=[]  CS8Rot=[]  CS9Pos=[]  CS9Rot=[]  CS10Pos=[]  CS10Rot=[]  CS11Pos=[]  CS11Rot=[]  CS12Pos=[]  CS12Rot=[]  CS13Pos=[]  CS13Rot=[]  CS14Pos=[]  CS14Rot=[]  CS15Pos=[]  CS15Rot=[]  CS16Pos=[]  CS16Rot=[]  CS17Pos=[]  CS17Rot=[]  CS18Pos=[]  CS18Rot=[]  CS19Pos=[]  CS19Rot=[]  CS20Pos=[]  CS20Rot=[]
  ZYLINDER-1 : mblibv1/Bodies/Body  DialogController=MECH.DynMechDlgSource  PhysicalDomain=mechanical  SubClassName=Unknown  LeftPortType=workingframe  RightPortType=workingframe  LConnTagsString=CS2  PMImportedID=19  UpdateFromCAD=on  DialogClass=MechanicalBodyBlock  Mass=1  MassUnits=kg  InertiaUnits=kg*m^2  Inertia=eye(3)  Shape=Cylinder  ShapeDims=[1 1]  ShapeUnits=m  ShapeUse=false  Density=1  DensityUnits=kg/m^3  DensityUse=false  GraphicsMode=CONVHULL  GraphicsFileName=ZYLINDER_prt.stl  BodyColorSelMode=MACHINE_DEFAULT  BodyColor=[1 0 0]  AttachedToCS=CS1  CG=Right$CG$[-25 46.5 0]$WORLD$WORLD$mm$[0 0 1;0 1 0;-1 0 0]$3x3 Transform$rad$WORLD$false$19::CG(AUTOGEN)  WorkingFrames=Right$CS1$[-25 46.5 0]$WORLD$WORLD$mm$[0 0 1;0 1 0;-1 0 0]$3x3 Transform$rad$WORLD$false$19::CS1(AUTOGEN)#Left$CS2$[-25 46.5 0]$WORLD$WORLD$mm$[1 0 0;0 1 0;0 0 1]$3x3 Transform$rad$WORLD$true$19:-:RootPart::19(AUTOGEN)  CGPos=[-25 46.5 0]  CGRot=[0 0 1;0 1 0;-1 0 0]  CS0Pos=[]  CS0Rot=[]  CS1Pos=[-25 46.5 0]  CS1Rot=[0 0 1;0 1 0;-1 0 0]  CS2Pos=[-25 46.5 0]  CS2Rot=[1 0 0;0 1 0;0 0 1]  CS3Pos=[]  CS3Rot=[]  CS4Pos=[]  CS4Rot=[]  CS5Pos=[]  CS5Rot=[]  CS6Pos=[]  CS6Rot=[]  CS7Pos=[]  CS7Rot=[]  CS8Pos=[]  CS8Rot=[]  CS9Pos=[]  CS9Rot=[]  CS10Pos=[]  CS10Rot=[]  CS11Pos=[]  CS11Rot=[]  CS12Pos=[]  CS12Rot=[]  CS13Pos=[]  CS13Rot=[]  CS14Pos=[]  CS14Rot=[]  CS15Pos=[]  CS15Rot=[]  CS16Pos=[]  CS16Rot=[]  CS17Pos=[]  CS17Rot=[]  CS18Pos=[]  CS18Rot=[]  CS19Pos=[]  CS19Rot=[]  CS20Pos=[]  CS20Rot=[]
  ZYLINDER-2 : mblibv1/Bodies/Body  DialogController=MECH.DynMechDlgSource  PhysicalDomain=mechanical  SubClassName=Unknown  LeftPortType=workingframe  RightPortType=workingframe  LConnTagsString=CS2  PMImportedID=30  UpdateFromCAD=on  DialogClass=MechanicalBodyBlock  Mass=0  MassUnits=kg  InertiaUnits=kg*m^2  Inertia=[0,0,0;0,0,0;0,0,0]  Shape=Cylinder  ShapeDims=[1 1]  ShapeUnits=m  ShapeUse=false  Density=1  DensityUnits=kg/m^3  DensityUse=false  GraphicsMode=GFXFILE  GraphicsFileName=ZYLINDER_prt.stl  BodyColorSelMode=MACHINE_DEFAULT  BodyColor=[1 0 0]  AttachedToCS=CS1  CG=Right$CG$[-25 14.3693 -44.2241]$WORLD$WORLD$mm$[0 0 1;-0.951057 0.309017 0;-0.309017 -0.951057 0]$3x3 Transform$rad$WORLD$false$30::CG(AUTOGEN)  WorkingFrames=Right$CS1$[-25 14.3693 -44.2241]$WORLD$WORLD$mm$[0 0 1;-0.951057 0.309017 0;-0.309017 -0.951057 0]$3x3 Transform$rad$WORLD$false$30::CS1(AUTOGEN)#Left$CS2$[-25 14.3693 -44.2241]$WORLD$WORLD$mm$[1 0 0;0 1 0;0 0 1]$3x3 Transform$rad$WORLD$true$30:-:RootPart::30(AUTOGEN)  CGPos=[-25 14.3693 -44.2241]  CGRot=[0 0 1;-0.951057 0.309017 0;-0.309017 -0.951057 0]  CS0Pos=[]  CS0Rot=[]  CS1Pos=[-25 14.3693 -44.2241]  CS1Rot=[0 0 1;-0.951057 0.309017 0;-0.309017 -0.951057 0]  CS2Pos=[-25 14.3693 -44.2241]  CS2Rot=[1 0 0;0 1 0;0 0 1]  CS3Pos=[]  CS3Rot=[]  CS4Pos=[]  CS4Rot=[]  CS5Pos=[]  CS5Rot=[]  CS6Pos=[]  CS6Rot=[]  CS7Pos=[]  CS7Rot=[]  CS8Pos=[]  CS8Rot=[]  CS9Pos=[]  CS9Rot=[]  CS10Pos=[]  CS10Rot=[]  CS11Pos=[]  CS11Rot=[]  CS12Pos=[]  CS12Rot=[]  CS13Pos=[]  CS13Rot=[]  CS14Pos=[]  CS14Rot=[]  CS15Pos=[]  CS15Rot=[]  CS16Pos=[]  CS16Rot=[]  CS17Pos=[]  CS17Rot=[]  CS18Pos=[]  CS18Rot=[]  CS19Pos=[]  CS19Rot=[]  CS20Pos=[]  CS20Rot=[]
  ZYLINDER-3 : mblibv1/Bodies/Body  DialogController=MECH.DynMechDlgSource  PhysicalDomain=mechanical  SubClassName=Unknown  LeftPortType=workingframe  RightPortType=workingframe  LConnTagsString=CS2  PMImportedID=63  UpdateFromCAD=on  DialogClass=MechanicalBodyBlock  Mass=0  MassUnits=kg  InertiaUnits=kg*m^2  Inertia=[0,0,0;0,0,0;0,0,0]  Shape=Cylinder  ShapeDims=[1 1]  ShapeUnits=m  ShapeUse=false  Density=1  DensityUnits=kg/m^3  DensityUse=false  GraphicsMode=GFXFILE  GraphicsFileName=ZYLINDER_prt.stl  BodyColorSelMode=MACHINE_DEFAULT  BodyColor=[1 0 0]  AttachedToCS=CS1  CG=Right$CG$[-25 14.3693 44.2241]$WORLD$WORLD$mm$[0 0 1;0.951057 0.309017 0;-0.309017 0.951057 0]$3x3 Transform$rad$WORLD$false$63::CG(AUTOGEN)  WorkingFrames=Right$CS1$[-25 14.3693 44.2241]$WORLD$WORLD$mm$[0 0 1;0.951057 0.309017 0;-0.309017 0.951057 0]$3x3 Transform$rad$WORLD$false$63::CS1(AUTOGEN)#Left$CS2$[-25 14.3693 44.2241]$WORLD$WORLD$mm$[1 0 0;0 1 0;0 0 1]$3x3 Transform$rad$WORLD$true$63:-:RootPart::63(AUTOGEN)  CGPos=[-25 14.3693 44.2241]  CGRot=[0 0 1;0.951057 0.309017 0;-0.309017 0.951057 0]  CS0Pos=[]  CS0Rot=[]  CS1Pos=[-25 14.3693 44.2241]  CS1Rot=[0 0 1;0.951057 0.309017 0;-0.309017 0.951057 0]  CS2Pos=[-25 14.3693 44.2241]  CS2Rot=[1 0 0;0 1 0;0 0 1]  CS3Pos=[]  CS3Rot=[]  CS4Pos=[]  CS4Rot=[]  CS5Pos=[]  CS5Rot=[]  CS6Pos=[]  CS6Rot=[]  CS7Pos=[]  CS7Rot=[]  CS8Pos=[]  CS8Rot=[]  CS9Pos=[]  CS9Rot=[]  CS10Pos=[]  CS10Rot=[]  CS11Pos=[]  CS11Rot=[]  CS12Pos=[]  CS12Rot=[]  CS13Pos=[]  CS13Rot=[]  CS14Pos=[]  CS14Rot=[]  CS15Pos=[]  CS15Rot=[]  CS16Pos=[]  CS16Rot=[]  CS17Pos=[]  CS17Rot=[]  CS18Pos=[]  CS18Rot=[]  CS19Pos=[]  CS19Rot=[]  CS20Pos=[]  CS20Rot=[]
  ZYLINDER-4 : mblibv1/Bodies/Body  DialogController=MECH.DynMechDlgSource  PhysicalDomain=mechanical  SubClassName=Unknown  LeftPortType=workingframe  RightPortType=workingframe  LConnTagsString=CS2  PMImportedID=90  UpdateFromCAD=on  DialogClass=MechanicalBodyBlock  Mass=0  MassUnits=kg  InertiaUnits=kg*m^2  Inertia=[0,0,0;0,0,0;0,0,0]  Shape=Cylinder  ShapeDims=[1 1]  ShapeUnits=m  ShapeUse=false  Density=1  DensityUnits=kg/m^3  DensityUse=false  GraphicsMode=GFXFILE  GraphicsFileName=ZYLINDER_prt.stl  BodyColorSelMode=MACHINE_DEFAULT  BodyColor=[1 0 0]  AttachedToCS=CS1  CG=Right$CG$[-25 -37.6193 27.332]$WORLD$WORLD$mm$[0 0 1;0.587785 -0.809017 0;0.809017 0.587785 0]$3x3 Transform$rad$WORLD$false$90::CG(AUTOGEN)  WorkingFrames=Right$CS1$[-25 -37.6193 27.332]$WORLD$WORLD$mm$[0 0 1;0.587785 -0.809017 0;0.809017 0.587785 0]$3x3 Transform$rad$WORLD$false$90::CS1(AUTOGEN)#Left$CS2$[-25 -37.6193 27.332]$WORLD$WORLD$mm$[1 0 0;0 1 0;0 0 1]$3x3 Transform$rad$WORLD$true$90:-:RootPart::90(AUTOGEN)  CGPos=[-25 -37.6193 27.332]  CGRot=[0 0 1;0.587785 -0.809017 0;0.809017 0.587785 0]  CS0Pos=[]  CS0Rot=[]  CS1Pos=[-25 -37.6193 27.332]  CS1Rot=[0 0 1;0.587785 -0.809017 0;0.809017 0.587785 0]  CS2Pos=[-25 -37.6193 27.332]  CS2Rot=[1 0 0;0 1 0;0 0 1]  CS3Pos=[]  CS3Rot=[]  CS4Pos=[]  CS4Rot=[]  CS5Pos=[]  CS5Rot=[]  CS6Pos=[]  CS6Rot=[]  CS7Pos=[]  CS7Rot=[]  CS8Pos=[]  CS8Rot=[]  CS9Pos=[]  CS9Rot=[]  CS10Pos=[]  CS10Rot=[]  CS11Pos=[]  CS11Rot=[]  CS12Pos=[]  CS12Rot=[]  CS13Pos=[]  CS13Rot=[]  CS14Pos=[]  CS14Rot=[]  CS15Pos=[]  CS15Rot=[]  CS16Pos=[]  CS16Rot=[]  CS17Pos=[]  CS17Rot=[]  CS18Pos=[]  CS18Rot=[]  CS19Pos=[]  CS19Rot=[]  CS20Pos=[]  CS20Rot=[]
  ZYL_BUCHSE : mblibv1/Bodies/Body  DialogController=MECH.DynMechDlgSource  PhysicalDomain=mechanical  SubClassName=Unknown  LeftPortType=workingframe  RightPortType=workingframe  LConnTagsString=CS2  RConnTagsString=CS3  PMImportedID=42  UpdateFromCAD=on  DialogClass=MechanicalBodyBlock  Mass=9.22021e+006  MassUnits=kg  InertiaUnits=kg*m^2  Inertia=[1649.68,0,0;0,2339.31,0;0,0,2306.91]  Shape=Cylinder  ShapeDims=[1 1]  ShapeUnits=m  ShapeUse=false  Density=1  DensityUnits=kg/m^3  DensityUse=false  GraphicsMode=GFXFILE  GraphicsFileName=ZYL_BUCHSE_prt.stl  BodyColorSelMode=MACHINE_DEFAULT  BodyColor=[1 0 0]  AttachedToCS=CS1  CG=Right$CG$[-25 -51.4707 -37.3957]$WORLD$WORLD$mm$[0 0 1;0.809017 -0.587785 0;0.587785 0.809017 0]$3x3 Transform$rad$WORLD$false$42::CG(AUTOGEN)  WorkingFrames=Right$CS1$[-25 -65.9098 -47.8863]$WORLD$WORLD$mm$[0 0 1;0.809017 -0.587785 0;0.587785 0.809017 0]$3x3 Transform$rad$WORLD$false$42::CS1(AUTOGEN)#Left$CS2$[-25 -51.4707 -37.3957]$WORLD$WORLD$mm$[1 0 0;0 1 0;0 0 1]$3x3 Transform$rad$WORLD$true$42:-:RootPart::42(AUTOGEN)#Right$CS3$[-25 -33.5491 -24.3749]$WORLD$WORLD$mm$[1 0 0;0 1 0;0 0 1]$3x3 Transform$rad$WORLD$true$106:-:42::42(AUTOGEN)  CGPos=[-25 -51.4707 -37.3957]  CGRot=[0 0 1;0.809017 -0.587785 0;0.587785 0.809017 0]  CS0Pos=[]  CS0Rot=[]  CS1Pos=[-25 -65.9098 -47.8863]  CS1Rot=[0 0 1;0.809017 -0.587785 0;0.587785 0.809017 0]  CS2Pos=[-25 -51.4707 -37.3957]  CS2Rot=[1 0 0;0 1 0;0 0 1]  CS3Pos=[-25 -33.5491 -24.3749]  CS3Rot=[1 0 0;0 1 0;0 0 1]  CS4Pos=[]  CS4Rot=[]  CS5Pos=[]  CS5Rot=[]  CS6Pos=[]  CS6Rot=[]  CS7Pos=[]  CS7Rot=[]  CS8Pos=[]  CS8Rot=[]  CS9Pos=[]  CS9Rot=[]  CS10Pos=[]  CS10Rot=[]  CS11Pos=[]  CS11Rot=[]  CS12Pos=[]  CS12Rot=[]  CS13Pos=[]  CS13Rot=[]  CS14Pos=[]  CS14Rot=[]  CS15Pos=[]  CS15Rot=[]  CS16Pos=[]  CS16Rot=[]  CS17Pos=[]  CS17Rot=[]  CS18Pos=[]  CS18Rot=[]  CS19Pos=[]  CS19Rot=[]  CS20Pos=[]  CS20Rot=[]
  ZYL_BUCHSE-1 : mblibv1/Bodies/Body  DialogController=MECH.DynMechDlgSource  PhysicalDomain=mechanical  SubClassName=Unknown  LeftPortType=workingframe  RightPortType=workingframe  LConnTagsString=CS2  RConnTagsString=CS3  PMImportedID=18  UpdateFromCAD=on  DialogClass=MechanicalBodyBlock  Mass=9.22021e+006  MassUnits=kg  InertiaUnits=kg*m^2  Inertia=[1649.68,0,0;0,2339.31,0;0,0,2306.91]  Shape=Cylinder  ShapeDims=[1 1]  ShapeUnits=m  ShapeUse=false  Density=1  DensityUnits=kg/m^3  DensityUse=false  GraphicsMode=GFXFILE  GraphicsFileName=ZYL_BUCHSE_prt.stl  BodyColorSelMode=MACHINE_DEFAULT  BodyColor=[1 0 0]  AttachedToCS=CS1  CG=Right$CG$[-25 63.6213 0]$WORLD$WORLD$mm$[0 0 1;-1 0 0;0 -1 0]$3x3 Transform$rad$WORLD$false$18::CG(AUTOGEN)  WorkingFrames=Right$CS1$[-25 81.469 0]$WORLD$WORLD$mm$[0 0 1;-1 0 0;0 -1 0]$3x3 Transform$rad$WORLD$false$18::CS1(AUTOGEN)#Left$CS2$[-25 63.6213 0]$WORLD$WORLD$mm$[1 0 0;0 1 0;0 0 1]$3x3 Transform$rad$WORLD$true$18:-:RootPart::18(AUTOGEN)#Right$CS3$[-25 41.469 0]$WORLD$WORLD$mm$[1 0 0;0 1 0;0 0 1]$3x3 Transform$rad$WORLD$true$18:-:73::18(AUTOGEN)  CGPos=[-25 63.6213 0]  CGRot=[0 0 1;-1 0 0;0 -1 0]  CS0Pos=[]  CS0Rot=[]  CS1Pos=[-25 81.469 0]  CS1Rot=[0 0 1;-1 0 0;0 -1 0]  CS2Pos=[-25 63.6213 0]  CS2Rot=[1 0 0;0 1 0;0 0 1]  CS3Pos=[-25 41.469 0]  CS3Rot=[1 0 0;0 1 0;0 0 1]  CS4Pos=[]  CS4Rot=[]  CS5Pos=[]  CS5Rot=[]  CS6Pos=[]  CS6Rot=[]  CS7Pos=[]  CS7Rot=[]  CS8Pos=[]  CS8Rot=[]  CS9Pos=[]  CS9Rot=[]  CS10Pos=[]  CS10Rot=[]  CS11Pos=[]  CS11Rot=[]  CS12Pos=[]  CS12Rot=[]  CS13Pos=[]  CS13Rot=[]  CS14Pos=[]  CS14Rot=[]  CS15Pos=[]  CS15Rot=[]  CS16Pos=[]  CS16Rot=[]  CS17Pos=[]  CS17Rot=[]  CS18Pos=[]  CS18Rot=[]  CS19Pos=[]  CS19Rot=[]  CS20Pos=[]  CS20Rot=[]
  ZYL_BUCHSE-2 : mblibv1/Bodies/Body  DialogController=MECH.DynMechDlgSource  PhysicalDomain=mechanical  SubClassName=Unknown  LeftPortType=workingframe  RightPortType=workingframe  LConnTagsString=CS2  RConnTagsString=CS3  PMImportedID=29  UpdateFromCAD=on  DialogClass=MechanicalBodyBlock  Mass=9.22021e+006  MassUnits=kg  InertiaUnits=kg*m^2  Inertia=[1649.68,0,0;0,2339.31,0;0,0,2306.91]  Shape=Cylinder  ShapeDims=[1 1]  ShapeUnits=m  ShapeUse=false  Density=1  DensityUnits=kg/m^3  DensityUse=false  GraphicsMode=GFXFILE  GraphicsFileName=ZYL_BUCHSE_prt.stl  BodyColorSelMode=MACHINE_DEFAULT  BodyColor=[1 0 0]  AttachedToCS=CS1  CG=Right$CG$[-25 19.6601 -60.5075]$WORLD$WORLD$mm$[0 0 1;-0.309017 -0.951057 0;0.951057 -0.309017 0]$3x3 Transform$rad$WORLD$false$29::CG(AUTOGEN)  WorkingFrames=Right$CS1$[-25 25.1753 -77.4816]$WORLD$WORLD$mm$[0 0 1;-0.309017 -0.951057 0;0.951057 -0.309017 0]$3x3 Transform$rad$WORLD$false$29::CS1(AUTOGEN)#Left$CS2$[-25 19.6601 -60.5075]$WORLD$WORLD$mm$[1 0 0;0 1 0;0 0 1]$3x3 Transform$rad$WORLD$true$29:-:RootPart::29(AUTOGEN)#Right$CS3$[-25 12.8146 -39.4393]$WORLD$WORLD$mm$[1 0 0;0 1 0;0 0 1]$3x3 Transform$rad$WORLD$true$29:-:75::29(AUTOGEN)  CGPos=[-25 19.6601 -60.5075]  CGRot=[0 0 1;-0.309017 -0.951057 0;0.951057 -0.309017 0]  CS0Pos=[]  CS0Rot=[]  CS1Pos=[-25 25.1753 -77.4816]  CS1Rot=[0 0 1;-0.309017 -0.951057 0;0.951057 -0.309017 0]  CS2Pos=[-25 19.6601 -60.5075]  CS2Rot=[1 0 0;0 1 0;0 0 1]  CS3Pos=[-25 12.8146 -39.4393]  CS3Rot=[1 0 0;0 1 0;0 0 1]  CS4Pos=[]  CS4Rot=[]  CS5Pos=[]  CS5Rot=[]  CS6Pos=[]  CS6Rot=[]  CS7Pos=[]  CS7Rot=[]  CS8Pos=[]  CS8Rot=[]  CS9Pos=[]  CS9Rot=[]  CS10Pos=[]  CS10Rot=[]  CS11Pos=[]  CS11Rot=[]  CS12Pos=[]  CS12Rot=[]  CS13Pos=[]  CS13Rot=[]  CS14Pos=[]  CS14Rot=[]  CS15Pos=[]  CS15Rot=[]  CS16Pos=[]  CS16Rot=[]  CS17Pos=[]  CS17Rot=[]  CS18Pos=[]  CS18Rot=[]  CS19Pos=[]  CS19Rot=[]  CS20Pos=[]  CS20Rot=[]
  ZYL_BUCHSE-3 : mblibv1/Bodies/Body  DialogController=MECH.DynMechDlgSource  PhysicalDomain=mechanical  SubClassName=Unknown  LeftPortType=workingframe  RightPortType=workingframe  LConnTagsString=CS2  RConnTagsString=CS3  PMImportedID=62  UpdateFromCAD=on  DialogClass=MechanicalBodyBlock  Mass=9.22021e+006  MassUnits=kg  InertiaUnits=kg*m^2  Inertia=[1649.68,0,0;0,2339.31,0;0,0,2306.91]  Shape=Cylinder  ShapeDims=[1 1]  ShapeUnits=m  ShapeUse=false  Density=1  DensityUnits=kg/m^3  DensityUse=false  GraphicsMode=GFXFILE  GraphicsFileName=ZYL_BUCHSE_prt.stl  BodyColorSelMode=MACHINE_DEFAULT  BodyColor=[1 0 0]  AttachedToCS=CS1  CG=Right$CG$[-25 19.6601 60.5075]$WORLD$WORLD$mm$[0 0 1;-0.309017 0.951057 0;-0.951057 -0.309017 0]$3x3 Transform$rad$WORLD$false$62::CG(AUTOGEN)  WorkingFrames=Right$CS1$[-25 25.1753 77.4816]$WORLD$WORLD$mm$[0 0 1;-0.309017 0.951057 0;-0.951057 -0.309017 0]$3x3 Transform$rad$WORLD$false$62::CS1(AUTOGEN)#Left$CS2$[-25 19.6601 60.5075]$WORLD$WORLD$mm$[1 0 0;0 1 0;0 0 1]$3x3 Transform$rad$WORLD$true$62:-:RootPart::62(AUTOGEN)#Right$CS3$[-25 12.8146 39.4393]$WORLD$WORLD$mm$[1 0 0;0 1 0;0 0 1]$3x3 Transform$rad$WORLD$true$110:-:62::62(AUTOGEN)  CGPos=[-25 19.6601 60.5075]  CGRot=[0 0 1;-0.309017 0.951057 0;-0.951057 -0.309017 0]  CS0Pos=[]  CS0Rot=[]  CS1Pos=[-25 25.1753 77.4816]  CS1Rot=[0 0 1;-0.309017 0.951057 0;-0.951057 -0.309017 0]  CS2Pos=[-25 19.6601 60.5075]  CS2Rot=[1 0 0;0 1 0;0 0 1]  CS3Pos=[-25 12.8146 39.4393]  CS3Rot=[1 0 0;0 1 0;0 0 1]  CS4Pos=[]  CS4Rot=[]  CS5Pos=[]  CS5Rot=[]  CS6Pos=[]  CS6Rot=[]  CS7Pos=[]  CS7Rot=[]  CS8Pos=[]  CS8Rot=[]  CS9Pos=[]  CS9Rot=[]  CS10Pos=[]  CS10Rot=[]  CS11Pos=[]  CS11Rot=[]  CS12Pos=[]  CS12Rot=[]  CS13Pos=[]  CS13Rot=[]  CS14Pos=[]  CS14Rot=[]  CS15Pos=[]  CS15Rot=[]  CS16Pos=[]  CS16Rot=[]  CS17Pos=[]  CS17Rot=[]  CS18Pos=[]  CS18Rot=[]  CS19Pos=[]  CS19Rot=[]  CS20Pos=[]  CS20Rot=[]
  ZYL_BUCHSE-4 : mblibv1/Bodies/Body  DialogController=MECH.DynMechDlgSource  PhysicalDomain=mechanical  SubClassName=Unknown  LeftPortType=workingframe  RightPortType=workingframe  LConnTagsString=CS2  RConnTagsString=CS3  PMImportedID=89  UpdateFromCAD=on  DialogClass=MechanicalBodyBlock  Mass=9.22021e+006  MassUnits=kg  InertiaUnits=kg*m^2  Inertia=[1649.68,0,0;0,2339.31,0;0,0,2306.91]  Shape=Cylinder  ShapeDims=[1 1]  ShapeUnits=m  ShapeUse=false  Density=1  DensityUnits=kg/m^3  DensityUse=false  GraphicsMode=GFXFILE  GraphicsFileName=ZYL_BUCHSE_prt.stl  BodyColorSelMode=MACHINE_DEFAULT  BodyColor=[1 0 0]  AttachedToCS=CS1  CG=Right$CG$[-25 -51.4707 37.3957]$WORLD$WORLD$mm$[0 0 1;0.809017 0.587785 0;-0.587785 0.809017 0]$3x3 Transform$rad$WORLD$false$89::CG(AUTOGEN)  WorkingFrames=Right$CS1$[-25 -65.9098 47.8863]$WORLD$WORLD$mm$[0 0 1;0.809017 0.587785 0;-0.587785 0.809017 0]$3x3 Transform$rad$WORLD$false$89::CS1(AUTOGEN)#Left$CS2$[-25 -51.4707 37.3957]$WORLD$WORLD$mm$[1 0 0;0 1 0;0 0 1]$3x3 Transform$rad$WORLD$true$89:-:RootPart::89(AUTOGEN)#Right$CS3$[-25 -33.5491 24.3749]$WORLD$WORLD$mm$[1 0 0;0 1 0;0 0 1]$3x3 Transform$rad$WORLD$true$81:-:89::89(AUTOGEN)  CGPos=[-25 -51.4707 37.3957]  CGRot=[0 0 1;0.809017 0.587785 0;-0.587785 0.809017 0]  CS0Pos=[]  CS0Rot=[]  CS1Pos=[-25 -65.9098 47.8863]  CS1Rot=[0 0 1;0.809017 0.587785 0;-0.587785 0.809017 0]  CS2Pos=[-25 -51.4707 37.3957]  CS2Rot=[1 0 0;0 1 0;0 0 1]  CS3Pos=[-25 -33.5491 24.3749]  CS3Rot=[1 0 0;0 1 0;0 0 1]  CS4Pos=[]  CS4Rot=[]  CS5Pos=[]  CS5Rot=[]  CS6Pos=[]  CS6Rot=[]  CS7Pos=[]  CS7Rot=[]  CS8Pos=[]  CS8Rot=[]  CS9Pos=[]  CS9Rot=[]  CS10Pos=[]  CS10Rot=[]  CS11Pos=[]  CS11Rot=[]  CS12Pos=[]  CS12Rot=[]  CS13Pos=[]  CS13Rot=[]  CS14Pos=[]  CS14Rot=[]  CS15Pos=[]  CS15Rot=[]  CS16Pos=[]  CS16Rot=[]  CS17Pos=[]  CS17Rot=[]  CS18Pos=[]  CS18Rot=[]  CS19Pos=[]  CS19Rot=[]  CS20Pos=[]  CS20Rot=[]
  wires:
  Constant/1 -> Joint Actuator/1
  Body Sensor1/1 -> Scope/1
  connections:
  RootPart/RConn1 -- Weld/LConn1
  Weld/RConn1 -- ZYL-KOPF/LConn1
  RootPart/RConn2 -- Weld1/LConn1
  Weld1/RConn1 -- ZYL-KOPF-1/LConn1
  RootPart/RConn3 -- Weld2/LConn1
  Weld2/RConn1 -- ZYL-KOPF-2/LConn1
  RootPart/RConn4 -- Weld3/LConn1
  Weld3/RConn1 -- ZYL-KOPF-3/LConn1
  RootPart/RConn5 -- Weld4/LConn1
  Weld4/RConn1 -- ZYL-KOPF-4/LConn1
  RootPart/RConn6 -- Weld5/LConn1
  Weld5/RConn1 -- ZYLINDER/LConn1
  RootPart/RConn7 -- Weld6/LConn1
  Weld6/RConn1 -- ZYLINDER-1/LConn1
  RootPart/RConn8 -- Weld7/LConn1
  Weld7/RConn1 -- ZYLINDER-2/LConn1
  RootPart/RConn9 -- Weld8/LConn1
  Weld8/RConn1 -- ZYLINDER-3/LConn1
  RootPart/RConn10 -- Weld9/LConn1
  Weld9/RConn1 -- ZYLINDER-4/LConn1
  RootPart/RConn11 -- Weld10/LConn1
  Weld10/RConn1 -- ZYL_BUCHSE/LConn1
  RootPart/RConn12 -- Weld11/LConn1
  Weld11/RConn1 -- ZYL_BUCHSE-1/LConn1
  RootPart/RConn13 -- Weld12/LConn1
  Weld12/RConn1 -- ZYL_BUCHSE-2/LConn1
  RootPart/RConn14 -- Weld13/LConn1
  Weld13/RConn1 -- ZYL_BUCHSE-3/LConn1
  RootPart/RConn15 -- Weld14/LConn1
  Weld14/RConn1 -- ZYL_BUCHSE-4/LConn1
  ZYL_BUCHSE-3/RConn1 -- Cylindrical/LConn1
  Cylindrical/RConn1 -- KOLBEN-3/LConn1
  ZYL_BUCHSE-4/RConn1 -- Cylindrical1/LConn1
  Cylindrical1/RConn1 -- KOLBEN-4/LConn1
  KURBELWELLE/RConn1 -- Cylindrical2/LConn1
  Cylindrical2/RConn1 -- HAUPT_PLEUEL/LConn1
  KURBELWELLE/RConn2 -- Weld15/LConn1
  Weld15/RConn1 -- PROPELLER/LConn1
  RootPart/RConn16 -- Revolute/LConn1
  Revolute/RConn1 -- KURBELWELLE/LConn1
  HAUPT_PLEUEL/RConn1 -- Revolute1/LConn1
  Revolute1/RConn1 -- PLEUEL/LConn1
  HAUPT_PLEUEL/RConn2 -- Revolute2/LConn1
  Revolute2/RConn1 -- PLEUEL-1/LConn1
  HAUPT_PLEUEL/RConn3 -- Revolute3/LConn1
  Revolute3/RConn1 -- PLEUEL-2/LConn1
  HAUPT_PLEUEL/RConn4 -- Revolute4/LConn1
  Revolute4/RConn1 -- PLEUEL-3/LConn1
  HAUPT_PLEUEL/RConn5 -- Cylindrical3/LConn1
  Cylindrical3/RConn1 -- KOLBEN-2/LConn1
  PLEUEL/RConn1 -- Cylindrical4/LConn1
  Cylindrical4/RConn1 -- KOLBEN/LConn1
  PLEUEL-1/RConn1 -- Cylindrical5/LConn1
  Cylindrical5/RConn1 -- KOLBEN-4/LConn2
  PLEUEL-2/RConn1 -- Cylindrical6/LConn1
  Cylindrical6/RConn1 -- KOLBEN-3/LConn2
  PLEUEL-3/RConn1 -- Cylindrical7/LConn1
  Cylindrical7/RConn1 -- KOLBEN-1/LConn1
  PROPELLER/RConn1 -- Weld16/LConn1
  Weld16/RConn1 -- SPINNER/LConn1
  ZYL_BUCHSE/RConn1 -- Cylindrical8/LConn1
  Cylindrical8/RConn1 -- KOLBEN/LConn2
  ZYL_BUCHSE-1/RConn1 -- Cylindrical9/LConn1
  Cylindrical9/RConn1 -- KOLBEN-1/LConn2
  ZYL_BUCHSE-2/RConn1 -- Cylindrical10/LConn1
  Cylindrical10/RConn1 -- KOLBEN-2/LConn2
  RootGround/RConn1 -- Weld17/LConn1
  Weld17/RConn1 -- RootPart/LConn1
  RootGround/LConn1 -- Machine Environment/RConn1
  Joint Actuator/RConn1 -- Cylindrical2/LConn2
  Body Sensor1/LConn1 -- PROPELLER/RConn2
